simulink library "outp"  (R2021b)
settings: Solver=VariableStepAuto  StartTime=0.0  StopTime=10.0  RelTol=1e-3
undefined symbols (not defined in the file or in its folder): ENUM_PMMMODE_CHARGE, ENUM_PMMMODE_IDLE, ENUM_PMMMODE_INITIALIZE, ENUM_PMMMODE_POWERDOWN, ENUM_PMMMODE_SLEEP, FALSE, Left, outp, slcm, TRUE
libraries: FVT_lib x956, hcu_lib x4, simulink x1
(part 5 of 10)

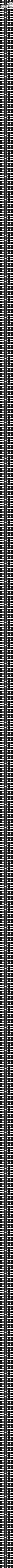
== system outp/OUTP/outpmodule ==
  VACC_EACEnDemand_enum : Inport
  VACC_CACTempOverHigh_flg : Inport  Port=2
  VACC_CACPresWarn_flg : Inport  Port=3
  VACC_CACPresReady_flg : Inport  Port=4
  VACC_EHPSEnDemand_enum : Inport  Port=5
  VACC_CACOverrun_flg : Inport  Port=6
  VACC_CACRunFail_flg : Inport  Port=7
  VACC_EHPSMotorDemSpd_rpm : Inport  Port=8
  VACC_EHPSSpdDemTimeout_flg : Inport  Port=9
  VACC_EHPSEnTimeout_flg : Inport  Port=10
  VACC_EHPSDisEnTimeout_flg : Inport  Port=11
  VACC_DCDCEnDemamd_enum : Inport  Port=12
  VACC_EHPSSpdCtrlMode_enum : Inport  Port=13
  VACC_EACSpdDemand_rpm : Inport  Port=14
  VACC_CACFanReq_flg : Inport  Port=15
  VAPM_VehSpeed_kph : Inport  Port=16
  VAPM_VehSpeedTimeOut_flg : Inport  Port=17
  VAPM_FSOffSw_enum : Inport  Port=18
  VAPM_FSOffSwTimeOut_flg : Inport  Port=19
  VAPM_ChrgPlugSta_enum : Inport  Port=20
  VAPM_PASDRMR_cm : Inport  Port=21
  VAPM_PASDRML_cm : Inport  Port=22
  VAPM_PASDRCR_cm : Inport  Port=23
  VAPM_PASDRCL_cm : Inport  Port=24
  VAPM_PASDFMR_cm : Inport  Port=25
  VAPM_PASDFML_cm : Inport  Port=26
  VAPM_PASDFCR_cm : Inport  Port=27
  VAPM_PASDFCL_cm : Inport  Port=28
  VAPM_APSDRLR_cm : Inport  Port=29
  VAPM_APSDRLL_cm : Inport  Port=30
  VAPM_APSDFLR_cm : Inport  Port=31
  VAPM_APSDFLL_cm : Inport  Port=32
  VAPM_PASAFCL_enum : Inport  Port=33
  VAPM_PASARMR_enum : Inport  Port=34
  VAPM_PASARML_enum : Inport  Port=35
  VAPM_PASARCR_enum : Inport  Port=36
  VAPM_PASARCL_enum : Inport  Port=37
  VAPM_PASAFMR_enum : Inport  Port=38
  VAPM_PASAFML_enum : Inport  Port=39
  VAPM_PASAFCR_enum : Inport  Port=40
  VAPM_USSStaRMR_flg : Inport  Port=41
  VAPM_USSStaRML_flg : Inport  Port=42
  VAPM_USSStaRLR_flg : Inport  Port=43
  VAPM_USSStaRLL_flg : Inport  Port=44
  VAPM_USSStaRCR_flg : Inport  Port=45
  VAPM_USSStaRCL_flg : Inport  Port=46
  VAPM_USSStaFMR_flg : Inport  Port=47
  VAPM_USSStaFML_flg : Inport  Port=48
  VAPM_USSStaFLR_flg : Inport  Port=49
  VAPM_USSStaFLL_flg : Inport  Port=50
  VAPM_USSStaFCR_flg : Inport  Port=51
  VAPM_USSStaFCL_flg : Inport  Port=52
  VAPM_Chime_enum : Inport  Port=53
  VAPM_SNSRLayout_enum : Inport  Port=54
  VAPM_StaFSya_flg : Inport  Port=55
  VAPM_ModOperation_enum : Inport  Port=56
  VAPM_BrkPedalPos_pct : Inport  Port=57
  VAPM_BrkPedalPosTimeOut_flg : Inport  Port=58
  VAPM_LFRawWhlSpeed_kph : Inport  Port=59
  VAPM_LFRawWhlSpeedTimeOut_flg : Inport  Port=60
  VAPM_RFRawWhlSpeed_kph : Inport  Port=61
  VAPM_RFRawWhlSpeedTimeOut_flg : Inport  Port=62
  VAPM_LRRawWhlSpeed_kph : Inport  Port=63
  VAPM_LRRawWhlSpeedTimeOut_flg : Inport  Port=64
  VAPM_RRRawWhlSpeed_kph : Inport  Port=65
  VAPM_RRRawWhlSpeedTimeOut_flg : Inport  Port=66
  VAPM_LFRawWhlSpeedV_flg : Inport  Port=67
  VAPM_LFRawWhlSpeedVTimeOut_flg : Inport  Port=68
  VAPM_RFRawWhlSpeedV_flg : Inport  Port=69
  VAPM_RFRawWhlSpeedVTimeOut_flg : Inport  Port=70
  VAPM_LRRawWhlSpeedV_flg : Inport  Port=71
  VAPM_LRRawWhlSpeedVTimeOut_flg : Inport  Port=72
  VAPM_RRRawWhlSpeedV_flg : Inport  Port=73
  VAPM_RRRawWhlSpeedVTimeOut_flg : Inport  Port=74
  VAPM_LFWhlRotDir_enum : Inport  Port=75
  VAPM_LFWhlRotDirTimeOut_flg : Inport  Port=76
  VAPM_RFWhlRotDir_enum : Inport  Port=77
  VAPM_RFWhlRotDirTimeOut_flg : Inport  Port=78
  VAPM_LRWhlRotDir_enum : Inport  Port=79
  VAPM_LRWhlRotDirTimeOut_flg : Inport  Port=80
  VAPM_RRWhlRotDir_enum : Inport  Port=81
  VAPM_RRWhlRotDirTimeOut_flg : Inport  Port=82
  VAPM_LFPulseCountV_flg : Inport  Port=83
  VAPM_LFPulseCountVTimeOut_flg : Inport  Port=84
  VAPM_RFPulseCountV_flg : Inport  Port=85
  VAPM_RFPulseCountVTimeOut_flg : Inport  Port=86
  VAPM_LRPulseCountV_flg : Inport  Port=87
  VAPM_LRPulseCountVTimeOut_flg : Inport  Port=88
  VAPM_RRPulseCountV_flg : Inport  Port=89
  VAPM_RRPulseCountVTimeOut_flg : Inport  Port=90
  VAPM_LFPulseCount_enum : Inport  Port=91
  VAPM_LFPulseCountTimeOut_flg : Inport  Port=92
  VAPM_RFPulseCount_enum : Inport  Port=93
  VAPM_RFPulseCountTimeOut_flg : Inport  Port=94
  VAPM_LRPulseCount_enum : Inport  Port=95
  VAPM_LRPulseCountTimeOut_flg : Inport  Port=96
  VAPM_RRPulseCount_enum : Inport  Port=97
  VAPM_RRPulseCountTimeOut_flg : Inport  Port=98
  VAPM_ShifterHandleCmd_enum : Inport  Port=99
  VAPM_ShifterHandleCmdTimeOut_flg : Inport  Port=100
  VAPM_DriIntend_enum : Inport  Port=101
  VAPM_DriIntendTimeOut_flg : Inport  Port=102
  VAPM_EPSAOIControl_enum : Inport  Port=103
  VAPM_EPSAOIControlTimeOut_flg : Inport  Port=104
  VAPM_SASAngle_Deg : Inport  Port=105
  VAPM_SASAngleTimeOut_flg : Inport  Port=106
  VAPM_SASSpeed_degps : Inport  Port=107
  VAPM_SASSpeedTimeOut_flg : Inport  Port=108
  VAPM_SASSpeedValid_flg : Inport  Port=109
  VAPM_SASSpeedValidTimeOut_flg : Inport  Port=110
  VAPM_SASCAL_flg : Inport  Port=111
  VAPM_SASCALTimeOut_flg : Inport  Port=112
  VAPM_SASV_flg : Inport  Port=113
  VAPM_SASVTimeOut_flg : Inport  Port=114
  VAPM_GRADE_Deg : Inport  Port=115
  VAPM_GRADETimeOut_flg : Inport  Port=116
  VAPM_YawRate_degps : Inport  Port=117
  VAPM_YawRateTimeOut_flg : Inport  Port=118
  VAPM_LatAccel_Gps : Inport  Port=119
  VAPM_LatAccelTimeOut_flg : Inport  Port=120
  VAPM_LongAccel_Gps : Inport  Port=121
  VAPM_LongAccelTimeOut_flg : Inport  Port=122
  VAPM_MCPressure_bar : Inport  Port=123
  VAPM_MCPressureTimeOut_flg : Inport  Port=124
  VAPM_YawRateV_flg : Inport  Port=125
  VAPM_YawRateVTimeOut_flg : Inport  Port=126
  VAPM_LatAccelV_flg : Inport  Port=127
  VAPM_LatAccelVTimeOut_flg : Inport  Port=128
  VAPM_LongAccelV_flg : Inport  Port=129
  VAPM_LongAccelVTimeOut_flg : Inport  Port=130
  VAPM_MCPressureV_bar : Inport  Port=131
  VAPM_MCPressureVTimeOut_flg : Inport  Port=132
  VAPM_BrkSwSta_flg : Inport  Port=133
  VAPM_BrkSwStaTimeOut_flg : Inport  Port=134
  VAPM_BrkSwV_flg : Inport  Port=135
  VAPM_BrkSwVTimeOut_flg : Inport  Port=136
  VAPM_ESCStandstill_flg : Inport  Port=137
  VAPM_ESCStandstillTimeOut_flg : Inport  Port=138
  VAPM_ESCAPSSta_enum : Inport  Port=139
  VAPM_ESCAPSStaTimeOut_flg : Inport  Port=140
  VAPM_EPBExtReleaseAvail_flg : Inport  Port=141
  VAPM_EPBExtReleaseAvailTimeOut_flg : Inport  Port=142
  VAPM_EPBExtApplyAvail_flg : Inport  Port=143
  VAPM_EPBExtApplyAvailTimeOut_flg : Inport  Port=144
  VAPM_EPBErrSta_enum : Inport  Port=145
  VAPM_EPBErrStaTimeOut_flg : Inport  Port=146
  VAPM_EPBSta_enum : Inport  Port=147
  VAPM_EPBStaTimeOut_flg : Inport  Port=148
  VAPM_AVMparkingcancel_enum : Inport  Port=149
  VAPM_AVMparkingcancelTimeOut_flg : Inport  Port=150
  VAPM_AVMparkingexcute_enum : Inport  Port=151
  VAPM_AVMparkingexcuteTimeOut_flg : Inport  Port=152
  VAPM_AVMParkingmode_enum : Inport  Port=153
  VAPM_AVMParkingmodeTimeOut_flg : Inport  Port=154
  VAPM_AVMErrSTA_flg : Inport  Port=155
  VAPM_AVMErrSTATimeOut_flg : Inport  Port=156
  VAPM_IVIStatus_flg : Inport  Port=157
  VAPM_IVIStatusTimeOut_flg : Inport  Port=158
  VAPM_CAASSw_enum : Inport  Port=159
  VAPM_CAASSwTimeOut_flg : Inport  Port=160
  VAPM_IVIScreen_enum : Inport  Port=161
  VAPM_IVIScreenTimeOut_flg : Inport  Port=162
  VAPM_ABSActive_flg : Inport  Port=163
  VAPM_ABSActiveTimeOut_flg : Inport  Port=164
  VAPM_TCSActive_flg : Inport  Port=165
  VAPM_TCSActiveTimeOut_flg : Inport  Port=166
  VAPM_DriverSeatBeltCmd_flg : Inport  Port=167
  VAPM_DriverSeatBeltCmdTimeOut_flg : Inport  Port=168
  VAPM_APSProgressPCT_pct : Inport  Port=169
  VAPM_APSRQDisplay_enum : Inport  Port=170
  VAPM_APSSWVer_enum : Inport  Port=171
  VAPM_APSHWVer_enum : Inport  Port=172
  VAPM_APSExitCondition_enum : Inport  Port=173
  VAPM_APSAngleTarget_Deg : Inport  Port=174
  VAPM_APSVRqEPASCtrl_flg : Inport  Port=175
  VAPM_APSRqEPASCtrl_flg : Inport  Port=176
  VAPM_CAASSta_enum : Inport  Port=177
  VAPM_DKCPDkeyAreaRAPSSta_enum : Inport  Port=178
  VAPM_DKCParkingModeCmd_enum : Inport  Port=179
  VAPM_PUIDLowPower_flg : Inport  Port=180
  VAPM_CAASVMCReqA_flg : Inport  Port=181
  VAPM_APSShiftPosnReq_enum : Inport  Port=182
  VAPM_APSSpeedCMD_kph : Inport  Port=183
  VAPM_APSVMCReqA_flg : Inport  Port=184
  VAPM_RAPSBCMLamp_enum : Inport  Port=185
  VAPM_RAPSBCMLockReq_flg : Inport  Port=186
  VAPM_APSPwrReq_enum : Inport  Port=187
  VAPM_RAPSErrWarnSta_enum : Inport  Port=188
  VAPM_RAPSErrLv1_flg : Inport  Port=189
  VAPM_IVIUserTakeOverAPSSta_flg : Inport  Port=190
  VBCM_FDCBCMLBeamCmd_flg : Inport  Port=191
  VBCM_FDCBCMPLampCmd_flg : Inport  Port=192
  VBCM_FDCBCMHBeamCmd_flg : Inport  Port=193
  VBCM_FDCBCMSMKLCmd_flg : Inport  Port=194
  VBCM_FDCBCMSMKRCmd_flg : Inport  Port=195
  VBCM_FDCBCMDVRSignalLCmd_flg : Inport  Port=196
  VBCM_FDCBCMDVRSignalRCmd_flg : Inport  Port=197
  VBCM_FDCBCMBSDBuzzerCmd_flg : Inport  Port=198
  VBCM_FDCBCMSLTLpCmd_flg : Inport  Port=199
  VBCM_FDCBCMSRTLpCmd_flg : Inport  Port=200
  VBCM_FDCBCMLTurnLpCmd_flg : Inport  Port=201
  VBCM_FDCBCMRTurnLpCmd_flg : Inport  Port=202
  VBCM_FDCBCMStopINDCmd_flg : Inport  Port=203
  VBCM_FDCBCMSTOPBALLCmd_flg : Inport  Port=204
  VBCM_FDCBCMInnerCallBellCmd_flg : Inport  Port=205
  VBCM_FDCBCMCallBellCmd_flg : Inport  Port=206
  VBCM_FDCBCMWiperHCmd_flg : Inport  Port=207
  VBCM_FDCBCMWasherCmd_flg : Inport  Port=208
  VBCM_FDCBCMWiperLCmd_flg : Inport  Port=209
  VBCM_FDCBCMLDRLCmd_flg : Inport  Port=210
  VBCM_FDCBCMRDRLCmd_flg : Inport  Port=211
  VBCM_FDCBCMRFLampCmd_flg : Inport  Port=212
  VBCM_TurnLpPatternSta_enum : Inport  Port=213
  VBCM_FDCBCMFDoorSta_flg : Inport  Port=214
  VBCM_FDCBCMMDoorSta_flg : Inport  Port=215
  VBCM_FDCBCMRDoorSta_flg : Inport  Port=216
  VBCM_FDCBCMRoomLpAmbCmd_flg : Inport  Port=217
  VBCM_FDCBCMLBSDRCmd_flg : Inport  Port=218
  VBCM_FDCBCMLBSDYCmd_flg : Inport  Port=219
  VBCM_FDCBCMRBSDRCmd_flg : Inport  Port=220
  VBCM_FDCBCMRBSDYCmd_flg : Inport  Port=221
  VBCM_FDCBCMEmExitSWSta_flg : Inport  Port=222
  VBCM_InnerBuzzerModeSta_enum : Inport  Port=223
  VBCM_FDCBCMInnerBuzzerCmd_flg : Inport  Port=224
  VBCM_FDCBCMRoomLpAmbSetSta_flg : Inport  Port=225
  VBCM_FDCBCMRoomLpSetSta_flg : Inport  Port=226
  VBCM_FDCBCMFRoomLpSetSta_pct : Inport  Port=227
  VBCM_FDCBCMFRoomLpCmd_pct : Inport  Port=228
  VBCM_FDCBCMMRoomLpSetSta_pct : Inport  Port=229
  VBCM_FDCBCMMRoomLpCmd_pct : Inport  Port=230
  VBCM_FDCBCMRRoomLpSetSta_pct : Inport  Port=231
  VBCM_FDCBCMRRoomLpCmd_pct : Inport  Port=232
  VBCM_FDCBCMHelpINDCmd_flg : Inport  Port=233
  VBCM_FDCBCMOSDrOpenSWSta_enum : Inport  Port=234
  VBCM_FDCBCMEmSVCmd_flg : Inport  Port=235
  VBCM_FDCBCMFDOpenSVCmd_flg : Inport  Port=236
  VBCM_FDCBCMFDCloseSVCmd_flg : Inport  Port=237
  VBCM_FDCBCMMDOpenSVCmd_flg : Inport  Port=238
  VBCM_FDCBCMMDCloseSVCmd_flg : Inport  Port=239
  VBCM_FDCBCMLTurnSWSta_flg : Inport  Port=240
  VBCM_FDCBCMRTurnSWSta_flg : Inport  Port=241
  VBCM_FDCBCMRGearSta_flg : Inport  Port=242
  VBCM_FDCBCMBrakeCmd_flg : Inport  Port=243
  VBCM_FDCBCMTurnBuzzerENSta_flg : Inport  Port=244
  VBCM_WakeUp_flg : Inport  Port=245
  VBCM_KeepWakeUp_flg : Inport  Port=246
  VDDM_C3BMS6RCDTC_raw32 : Inport  Port=247
  VDDM_C3BMS6CSDTC_raw32 : Inport  Port=248
  VDDM_C3BMS6LCDTC_raw32 : Inport  Port=249
  VDDM_C3BMS1RCDTC_raw32 : Inport  Port=250
  VDDM_C3BMS1CSDTC_raw32 : Inport  Port=251
  VDDM_C3BMS1LCDTC_raw32 : Inport  Port=252
  VDDM_C3CCU1RCDTC_raw32 : Inport  Port=253
  VDDM_C3CCU1CSDTC_raw32 : Inport  Port=254
  VDDM_C3CCU1LCDTC_raw32 : Inport  Port=255
  VDDM_C3CCU2RCDTC_raw32 : Inport  Port=256
  VDDM_C3CCU2CSDTC_raw32 : Inport  Port=257
  VDDM_C3CCU2LCDTC_raw32 : Inport  Port=258
  VDDM_C1ABM1RCDTC_raw32 : Inport  Port=259
  VDDM_C1ABM1CSDTC_raw32 : Inport  Port=260
  VDDM_C1ABM1LCDTC_raw32 : Inport  Port=261
  VDDM_Lv1ErrDTC_raw32 : Inport  Port=262
  VDDM_Lv2ErrDTC_raw32 : Inport  Port=263
  VDDM_Lv3ErrDTC_raw32 : Inport  Port=264
  VDDM_Lv4ErrDTC_raw32 : Inport  Port=265
  VDDM_BrkSWErrDTC_raw32 : Inport  Port=266
  VDDM_BrkSWNoBacDTC_raw32 : Inport  Port=267
  VDDM_KeyAuthDTC_raw32 : Inport  Port=268
  VDDM_ONtoRdyDTC_raw32 : Inport  Port=269
  VDDM_HVB4PreDTC_raw32 : Inport  Port=270
  VDDM_MCU4PreDTC_raw32 : Inport  Port=271
  VDDM_DCDC4PreDTC_raw32 : Inport  Port=272
  VDDM_HVRlyCloDTC_raw32 : Inport  Port=273
  VDDM_BMSRdyDTC_raw32 : Inport  Port=274
  VDDM_DCDCEnaDTC_raw32 : Inport  Port=275
  VDDM_HiLvSaChkDTC_raw32 : Inport  Port=276
  VDDM_MidLvSaChkDTC_raw32 : Inport  Port=277
  VDDM_MCUDisDTC_raw32 : Inport  Port=278
  VDDM_DCDCDisDTC_raw32 : Inport  Port=279
  VDDM_HVRlyOpDTC_raw32 : Inport  Port=280
  VDDM_MCUActDTC_raw32 : Inport  Port=281
  VDDM_OBC4PreDTC_raw32 : Inport  Port=282
  VDDM_IniLVLoDTC_raw32 : Inport  Port=283
  VDDM_LVSupLoDTC_raw32 : Inport  Port=284
  VDDM_LVSupHiDTC_raw32 : Inport  Port=285
  VDDM_DrStSWDTC_raw32 : Inport  Port=286
  VDDM_FLDoorSWDTC_raw32 : Inport  Port=287
  VDDM_RLDoorSWDTC_raw32 : Inport  Port=288
  VDDM_FRDoorSWDTC_raw32 : Inport  Port=289
  VDDM_RRDoorSWDTC_raw32 : Inport  Port=290
  VDDM_HoodSWDTC_raw32 : Inport  Port=291
  VDDM_TailgaSWDTC_raw32 : Inport  Port=292
  VDDM_EDriveSysErrVCUErr_flg : Inport  Port=293
  VDDM_VehMalfunLevel_enum : Inport  Port=294
  VDDM_APS1SigOoRDTC_raw32 : Inport  Port=295
  VDDM_APS2SigOoRDTC_raw32 : Inport  Port=296
  VDDM_APSCorrErrDTC_raw32 : Inport  Port=297
  VDDM_MCUF1NoComDTC_raw32 : Inport  Port=298
  VDDM_MCUR1NoComDTC_raw32 : Inport  Port=299
  VDDM_Shifter1NoComDTC_raw32 : Inport  Port=300
  VDDM_ESC7NoComDTC_raw32 : Inport  Port=301
  VDDM_ESC1NoComDTC_raw32 : Inport  Port=302
  VDDM_ESC5NoComDTC_raw32 : Inport  Port=303
  VDDM_EnterNewOperCyc_flg : Inport  Port=304
  VDDM_DiagHCrashDTC_raw32 : Inport  Port=305
  VDDM_DiagFLTSDTC_raw32 : Inport  Port=306
  VDDM_DiagFRTSDTC_raw32 : Inport  Port=307
  VDDM_DiagRLTSDTC_raw32 : Inport  Port=308
  VDDM_DiagRRTSDTC_raw32 : Inport  Port=309
  VDDM_FCLUSSDTC_raw32 : Inport  Port=310
  VDDM_FMLUSSDTC_raw32 : Inport  Port=311
  VDDM_FMRUSSDTC_raw32 : Inport  Port=312
  VDDM_FCRUSSDTC_raw32 : Inport  Port=313
  VDDM_RCLUSSDTC_raw32 : Inport  Port=314
  VDDM_RMLUSSDTC_raw32 : Inport  Port=315
  VDDM_RMRUSSDTC_raw32 : Inport  Port=316
  VDDM_RCRUSSDTC_raw32 : Inport  Port=317
  VDDM_FLLUSSDTC_raw32 : Inport  Port=318
  VDDM_FLRUSSDTC_raw32 : Inport  Port=319
  VDDM_RLLUSSDTC_raw32 : Inport  Port=320
  VDDM_RLRUSSDTC_raw32 : Inport  Port=321
  VDDM_FCM2NoComDTC_raw32 : Inport  Port=322
  VDDM_FCM2RCErrDTC_raw32 : Inport  Port=323
  VDDM_FCM2CSErrDTC_raw32 : Inport  Port=324
  VDDM_FCM3NoComDTC_raw32 : Inport  Port=325
  VDDM_FCM3RCErrDTC_raw32 : Inport  Port=326
  VDDM_FCM3CSErrDTC_raw32 : Inport  Port=327
  VDDM_FCM4NoComDTC_raw32 : Inport  Port=328
  VDDM_FCM4CSErrDTC_raw32 : Inport  Port=329
  VDDM_FCM5NoComDTC_raw32 : Inport  Port=330
  VDDM_FCM5CSErrDTC_raw32 : Inport  Port=331
  VDDM_ZoneSCPNoComDTC_raw32 : Inport  Port=332
  VDDM_BMSSigErrDetDTC_raw32 : Inport  Port=333
  VDDM_FCMACCSigErrDetDTC_raw32 : Inport  Port=334
  VDDM_FrMCUSigErrDetDTC_raw32 : Inport  Port=335
  VDDM_RrMCUSigErrDetDTC_raw32 : Inport  Port=336
  VDDM_CCUSigErrDetDTC_raw32 : Inport  Port=337
  VDDM_ACCAccelCmdErrDetDTC_raw32 : Inport  Port=338
  VDDM_ACCMalfuncDetDTC_raw32 : Inport  Port=339
  VDDM_CCMalfuncDetDTC_raw32 : Inport  Port=340
  VDDM_MSAMalfuncDetDTC_raw32 : Inport  Port=341
  VDDM_ISAMalfuncDetDTC_raw32 : Inport  Port=342
  VDDM_MCUF1RCErrDTC_raw32 : Inport  Port=343
  VDDM_MCUR1RCErrDTC_raw32 : Inport  Port=344
  VDDM_MCUF1CSErrDTC_raw32 : Inport  Port=345
  VDDM_MCUR1CSErrDTC_raw32 : Inport  Port=346
  VDDM_Shifter1RCErrDTC_raw32 : Inport  Port=347
  VDDM_Shifter1CSErrDTC_raw32 : Inport  Port=348
  VDDM_ESC7RCErrDTC_raw32 : Inport  Port=349
  VDDM_ESC7CSErrDTC_raw32 : Inport  Port=350
  VDDM_ESC1RCErrDTC_raw32 : Inport  Port=351
  VDDM_ESC1CSErrDTC_raw32 : Inport  Port=352
  VDDM_ESC5RCErrDTC_raw32 : Inport  Port=353
  VDDM_ESC5CSErrDTC_raw32 : Inport  Port=354
  VDDM_FrMCUTqErrDTC_raw32 : Inport  Port=355
  VDDM_RrMCUTqErrDTC_raw32 : Inport  Port=356
  VDDM_LFBatwarnDTC_raw32 : Inport  Port=357
  VDDM_RFBatwarnDTC_raw32 : Inport  Port=358
  VDDM_LRBatwarnDTC_raw32 : Inport  Port=359
  VDDM_RRBatwarnDTC_raw32 : Inport  Port=360
  VDDM_LFPressIndiDTC_raw32 : Inport  Port=361
  VDDM_RFPressIndiDTC_raw32 : Inport  Port=362
  VDDM_LRPressIndiDTC_raw32 : Inport  Port=363
  VDDM_RRPressIndiDTC_raw32 : Inport  Port=364
  VDDM_LFWheelTmpHighDTC_raw32 : Inport  Port=365
  VDDM_RFWheelTmpHighDTC_raw32 : Inport  Port=366
  VDDM_LRWheelTmpHighDTC_raw32 : Inport  Port=367
  VDDM_RRWheelTmpHighDTC_raw32 : Inport  Port=368
  VDDM_LFSensorFailDTC_raw32 : Inport  Port=369
  VDDM_RFSensorFailDTC_raw32 : Inport  Port=370
  VDDM_LRSensorFailDTC_raw32 : Inport  Port=371
  VDDM_RRSensorFailDTC_raw32 : Inport  Port=372
  VDDM_C1EPAS2LCDTC_raw32 : Inport  Port=373
  VDDM_5vAPS1PwrErrDTC_raw32 : Inport  Port=374
  VDDM_5vAPS2PwrErrDTC_raw32 : Inport  Port=375
  VDDM_EPBLockTODTC_raw32 : Inport  Port=376
  VDDM_EPBUnlockTODTC_raw32 : Inport  Port=377
  VDDM_LimpHomeActTmp_flg : Inport  Port=378
  VDDM_DTCDetect_enum : Inport  Port=379
  VDDM_EngagePFail_flg : Inport  Port=380
  VDDM_DisengagePFail_flg : Inport  Port=381
  VDDM_VCURAPSErrLv2_flg : Inport  Port=382
  VDDM_VCURAPSErrLv3_flg : Inport  Port=383
  VDDM_EDriveSysErrShifterErr_flg : Inport  Port=384
  VDDM_LVSysErrPwrOutErr_flg : Inport  Port=385
  VDDM_HVRlyOpFail_flg : Inport  Port=386
  VDDM_MCUActDisFail_flg : Inport  Port=387
  VDDM_VCUBrkSWSta_enum : Inport  Port=388
  VDDM_VCUFLDoorSta_flg : Inport  Port=389
  VDDM_VCUFRDoorSta_flg : Inport  Port=390
  VDDM_VCURLDoorSta_flg : Inport  Port=391
  VDDM_VCURRDoorSta_flg : Inport  Port=392
  VDDM_SysAllowReadySta_flg : Inport  Port=393
  VDDM_VCUHoodSWSta_flg : Inport  Port=394
  VDDM_VCUTailgateSWSta_flg : Inport  Port=395
  VDHP_ActAPSPosn_pct : Inport  Port=396
  VDHP_EAPS1MIN_pct : Inport  Port=397
  VDHP_EAPS2MIN_pct : Inport  Port=398
  VDHP_ResetPedalZeroPosStart_flg : Inport  Port=399
  VDHP_EAPS1NRM_pct : Inport  Port=400
  VDHP_EAPS2NRM_pct : Inport  Port=401
  VDID_VSS_kph : Inport  Port=402
  VDID_RUNTM_s : Inport  Port=403
  VDID_MILDIST_km : Inport  Port=404
  VDID_WARMUPS_cnt : Inport  Port=405
  VDID_CLRDIST_km : Inport  Port=406
  VDID_APPD_pct : Inport  Port=407
  VDID_APPE_pct : Inport  Port=408
  VDID_MILTIME_min : Inport  Port=409
  VDID_CLRTIME_min : Inport  Port=410
  VDID_BATSOC_pct : Inport  Port=411
  VDID_HEVBATT_V : Inport  Port=412
  VDID_ODOMETER_km : Inport  Port=413
  VDID_BATSOH_pct : Inport  Port=414
  VDID_HVBCellVoltMin_V : Inport  Port=415
  VDID_HVBCellVoltMax_V : Inport  Port=416
  VDID_HVESSCHARGELIM_kW : Inport  Port=417
  VDID_HVESSCHARGEACT_kW : Inport  Port=418
  VDID_HVESSENER_Whps : Inport  Port=419
  VDID_NUMPSATRIPSFLTMEMCLR_cnt : Inport  Port=420
  VDID_HVBattCurr_Ahps : Inport  Port=421
  VDID_PSAR_sec : Inport  Port=422
  VDID_PSAL_sec : Inport  Port=423
  VDID_IPSAR_sec : Inport  Port=424
  VDID_IPSAL_sec : Inport  Port=425
  VDID_CPSAR_sec : Inport  Port=426
  VDID_CPSAL_sec : Inport  Port=427
  VDID_HVBNAH_Ahr : Inport  Port=428
  VDID_HVBNE_kWh : Inport  Port=429
  VDID_IGNCNTR_cnt : Inport  Port=430
  VDID_TNBCPSAR_Ahr : Inport  Port=431
  VDID_TNBCPSAL_Ahr : Inport  Port=432
  VDID_TNECPSAR_kWh : Inport  Port=433
  VDID_TNECPSAL_kWh : Inport  Port=434
  VDID_TEBPSAR_kWh : Inport  Port=435
  VDID_TEBPSAL_kWh : Inport  Port=436
  VDID_TGEOVCR_kWh : Inport  Port=437
  VDID_TGEOVCL_kWh : Inport  Port=438
  VDID_GECHGOVCDCR_kWh : Inport  Port=439
  VDID_GECHGOVCDCL_kWh : Inport  Port=440
  VDID_GECHGOVCACR_kWh : Inport  Port=441
  VDID_GECHGOVCACL_kWh : Inport  Port=442
  VDID_RESSV2XENNONPSAR_kWh : Inport  Port=443
  VDID_RESSV2XENNONPSAL_kWh : Inport  Port=444
  VDID_PKER_kphsqr : Inport  Port=445
  VDID_PKEL_kphsqr : Inport  Port=446
  VDID_ResetCDEODTR_km : Inport  Port=447
  VDID_CDEODTR_km : Inport  Port=448
  VDID_CDEODTL_km : Inport  Port=449
  VDID_AvgBattTempPSAR_C : Inport  Port=450
  VDID_AvgBattTempPSAL_C : Inport  Port=451
  VDID_AvgBattTempOVCR_C : Inport  Port=452
  VDID_AvgBattTempOVCL_C : Inport  Port=453
  VDID_AvgBattTempOFFR_C : Inport  Port=454
  VDID_AvgBattTempOFFL_C : Inport  Port=455
  VDID_QTYPSATRIPSR_cnt : Inport  Port=456
  VDID_QTYPSATRIPSL_cnt : Inport  Port=457
  VDID_RESSCNTDODRNGR_cnt : Inport  Port=458
  VDID_RESSCNTDODRNGL_cnt : Inport  Port=459
  VDID_ETMATOER_kWh : Inport  Port=460
  VDID_ETMATOEL_kWh : Inport  Port=461
  VDID_ETMBTOER_kWh : Inport  Port=462
  VDID_ETMBTOEL_kWh : Inport  Port=463
  VDID_RESSTIMESOCPSARNGR_s : Inport  Port=464
  VDID_RESSTIMESOCPSARNGL_s : Inport  Port=465
  VDID_RESSTIMESOCCHGRNGR_s : Inport  Port=466
  VDID_RESSTIMESOCCHGRNGL_s : Inport  Port=467
  VDID_RESSTIMESOCOFFRNGR_s : Inport  Port=468
  VDID_RESSTIMESOCOFFRNGL_s : Inport  Port=469
  VDID_MAXBATTEMPL_C : Inport  Port=470
  VDID_MINBATTEMPL_C : Inport  Port=471
  VDID_AVGBATTEMPL_C : Inport  Port=472
  VDID_PROTOCOLID_enum : Inport  Port=473
  VDID_RESSTTEMPRNGAXIS_enum : Inport  Port=474
  VDID_RESSTIMESOCRNGAXIS_enum : Inport  Port=475
  VDID_RESSCNTSDODRNGAXIS_enum : Inport  Port=476
  VDID_CALID_cnt : Inport  Port=477
  VDID_ECUNAME_cnt : Inport  Port=478
  VDID_PKERNumerator_kphsqr : Inport  Port=479
  VDID_PKELNumerator_kphsqr : Inport  Port=480
  VDID_BattTempPSAR_sec : Inport  Port=481
  VDID_BattTempPSAL_sec : Inport  Port=482
  VDID_OVCR_sec : Inport  Port=483
  VDID_OVCL_sec : Inport  Port=484
  VDID_OFFR_sec : Inport  Port=485
  VDID_OFFL_sec : Inport  Port=486
  VDID_AVGBATTEMPL_sec : Inport  Port=487
  VDID_VinCode_cnt : Inport  Port=488
  VDID_STASUP_enum : Inport  Port=489
  VDID_HEVMODE_enum : Inport  Port=490
  VDID_HVBATT_A : Inport  Port=491
  VDID_DIDModelVersion_raw : Inport  Port=492
  VDID_DIDModelVersionChksum_raw : Inport  Port=493
  VDKC_DKCTimeSN_cnt : Inport  Port=494
  VDKC_DKCAuthSta_enum : Inport  Port=495
  VDKC_TimeSNDKCFbk_cnt : Inport  Port=496
  VDKC_KeyMissSta_flg : Inport  Port=497
  VDKC_KeyModeSta_enum : Inport  Port=498
  VDKC_DkeyShowIVISta_enum : Inport  Port=499
  VDKC_KeyAreaPS_enum : Inport  Port=500
  VDKC_KeyAreaLockUnlock_enum : Inport  Port=501
  VDKC_PCommandToBCM_enum : Inport  Port=502
  VDKC_DKeyWelcomeSta_enum : Inport  Port=503
  VDKC_KeyAreaPTG_enum : Inport  Port=504
  VDKC_KeyAreaSPTGSta_enum : Inport  Port=505
  VDKC_UIDLowPowerSta_enum : Inport  Port=506
  VDKC_DkeyAreaRAPSSta_enum : Inport  Port=507
  VDKC_ParkingModeCmd_enum : Inport  Port=508
  VDKC_KeyNumSta_enum : Inport  Port=509
  VDKC_KeyTypeSta_enum : Inport  Port=510
  VDKC_FDCDKCAllowSleep_flg : Inport  Port=511
  VDKC_JudgeKeepUnlockZone_flg : Inport  Port=512
  VDSC_DISCTurn_flg : Inport  Port=513
  VDSC_DISCTargetSpd_kph : Inport  Port=514
  VDSC_DISCSta_enum : Inport  Port=515
  VDSC_DISCButtSta_flg : Inport  Port=516
  VNMM_AllCANTxReq_flg : Inport  Port=517
  VNMM_NMmTxReq_flg : Inport  Port=518
  VNMM_Awake_enum : Inport  Port=519
  VNMM_CSB_flg : Inport  Port=520
  VNMM_ErrorState_enum : Inport  Port=521
  VNMM_NodeID_enum : Inport  Port=522
  VNMM_PNI_flg : Inport  Port=523
  VNMM_RptMsgReq_flg : Inport  Port=524
  VNMM_WakeUp_enum : Inport  Port=525
  VNMM_ActiveWU_flg : Inport  Port=526
  VNMM_SysNMmSta_enum : Inport  Port=527
  VNMM_NetworkReq_flg : Inport  Port=528
  VPMM_SysPowerMode_enum : Inport  Port=529
  VPMM_PowerUpState_enum : Inport  Port=530
  VPMM_PowerDownState_enum : Inport  Port=531
  VPMM_ChrgState_enum : Inport  Port=532
  VPMM_PowerUpFault_enum : Inport  Port=533
  VPMM_PowerDownFault_enum : Inport  Port=534
  VPMM_ChrgFault_enum : Inport  Port=535
  VPMM_IRCRlyClose_flg : Inport  Port=536
  VPMM_IGNRlyClose_flg : Inport  Port=537
  VPMM_BattHVDem_enum : Inport  Port=538
  VPMM_DCDCRlyDem_enum : Inport  Port=539
  VPMM_CACRlyDem_enum : Inport  Port=540
  VPMM_MCUHVLoopDem_enum : Inport  Port=541
  VPMM_EHPSRlyDem_enum : Inport  Port=542
  VPMM_ACHVLoopDem_enum : Inport  Port=543
  VPMM_HVSysReady_enum : Inport  Port=544
  VPMM_DrivelineRelease_enum : Inport  Port=545
  VPMM_ActiveDischargeReq_enum : Inport  Port=546
  VPMM_VCUMCUEn_flg : Inport  Port=547
  VPMM_VCUMCUFailRst_flg : Inport  Port=548
  VPMM_HVILFail_flg : Inport  Port=549
  VPMM_LostHVComActivePwrDown_flg : Inport  Port=550
  VPMM_LVBattLowInd_enum : Inport  Port=551
  VPMM_ChrgPowerUpFail_flg : Inport  Port=552
  VPMM_ChrgBCUHVFail_flg : Inport  Port=553
  VPMM_HVFailureChkPass_flg : Inport  Port=554
  VPMM_HVILDetectFail_flg : Inport  Port=555
  VPMM_V2BLifeSig_cnt : Inport  Port=556
  VPMM_V2BAux1OnOff_enum : Inport  Port=557
  VPMM_V2BAux2OnOff_enum : Inport  Port=558
  VPMM_V2BAux3OnOff_enum : Inport  Port=559
  VPMM_V2BMainPosRlySta_enum : Inport  Port=560
  VPMM_V2BMainPosRlyFit_enum : Inport  Port=561
  VPMM_V2BACPosRlySta_enum : Inport  Port=562
  VPMM_V2BACPosRlyFit_enum : Inport  Port=563
  VPMM_V2BAirPosRlySta_enum : Inport  Port=564
  VPMM_V2BAirPosRlyFit_enum : Inport  Port=565
  VPMM_V2BOilPosRlySta_enum : Inport  Port=566
  VPMM_V2BOilPosRlyFit_enum : Inport  Port=567
  VPMM_V2BDCDCPosRlySta_enum : Inport  Port=568
  VPMM_V2BDCDCPosRlyFit_enum : Inport  Port=569
  VPMM_V2BAux1RlySta_enum : Inport  Port=570
  VPMM_V2BAux1RlyFit_enum : Inport  Port=571
  VPMM_V2BAux2RlySta_enum : Inport  Port=572
  VPMM_V2BAux2RlyFit_enum : Inport  Port=573
  VPMM_V2BAux3RlySta_enum : Inport  Port=574
  VPMM_V2BAux3RlyFit_enum : Inport  Port=575
  VPMM_V2BAux4RlySta_enum : Inport  Port=576
  VPMM_V2BAux4RlyFit_enum : Inport  Port=577
  VPMM_VCULife1_cnt : Inport  Port=578
  VPMM_VCULife2_cnt : Inport  Port=579
  VPMM_VSPFunc_enum : Inport  Port=580
  VPMM_VSPIGNKeySta_enum : Inport  Port=581
  VPMM_VSPReversed_flg : Inport  Port=582
  VPMM_VSPTurnRight_enum : Inport  Port=583
  VPMM_VSPTurnLeft_enum : Inport  Port=584
  VPMM_FogTMSRlyCMD_enum : Inport  Port=585
  VPMM_DCCurr_A : Inport  Port=586
  VPMM_DCVol_V : Inport  Port=587
  VPSA_Keystatus_enum : Inport  Port=588
  VPSA_EmergencyShutDown_flg : Inport  Port=589
  VSCP_triggerBAM_flg : Inport  Port=590
  VSCP_CFGEM1Ctrl_raw : Inport  Port=591
  VSCP_CFGEM1BAMTSize_raw : Inport  Port=592
  VSCP_CFGEM1BAMTNum_raw : Inport  Port=593
  VSCP_CFGEM1BAMRsv_raw : Inport  Port=594
  VSCP_CFGEM1BAMPGN_raw : Inport  Port=595
  VSCP_triggerDT_flg : Inport  Port=596
  VSCP_DTbyte0_raw : Inport  Port=597
  VSCP_DTbyte1_raw : Inport  Port=598
  VSCP_DTbyte2_raw : Inport  Port=599
  VSCP_DTbyte3_raw : Inport  Port=600
  VSCP_DTbyte4_raw : Inport  Port=601
  VSCP_DTbyte5_raw : Inport  Port=602
  VSCP_DTbyte6_raw : Inport  Port=603
  VSCP_DTbyte7_raw : Inport  Port=604
  VSYS_HWVer1_cnt : Inport  Port=605
  VSYS_HWVer2_cnt : Inport  Port=606
  VSYS_HWVer3_cnt : Inport  Port=607
  VSYS_CarModel1_cnt : Inport  Port=608
  VSYS_CarModel2_cnt : Inport  Port=609
  VSYS_CarModel3_cnt : Inport  Port=610
  VSYS_ECU1_cnt : Inport  Port=611
  VSYS_ECU2_cnt : Inport  Port=612
  VSYS_Major1_cnt : Inport  Port=613
  VSYS_Major2_cnt : Inport  Port=614
  VSYS_Minor1_cnt : Inport  Port=615
  VSYS_Minor2_cnt : Inport  Port=616
  VSYS_Patch1_cnt : Inport  Port=617
  VSYS_Patch2_cnt : Inport  Port=618
  VSYS_Country1_cnt : Inport  Port=619
  VSYS_Country2_cnt : Inport  Port=620
  VSYS_Variation_cnt : Inport  Port=621
  VSYS_Dash1_cnt : Inport  Port=622
  VSYS_Change1_cnt : Inport  Port=623
  VSYS_Change2_cnt : Inport  Port=624
  VSYS_Dash2_cnt : Inport  Port=625
  VSYS_SHA1_cnt : Inport  Port=626
  VSYS_SHA2_cnt : Inport  Port=627
  VSYS_SHA3_cnt : Inport  Port=628
  VSYS_SHA4_cnt : Inport  Port=629
  VSYS_SHA5_cnt : Inport  Port=630
  VSYS_SHA6_cnt : Inport  Port=631
  VSYS_SHA7_cnt : Inport  Port=632
  VSYS_SHA8_cnt : Inport  Port=633
  VSYS_NvWriteReqRisingEdge_flg : Inport  Port=634
  VSYS_FdcSlpReqRisingEdge_flg : Inport  Port=635
  VSYS_FdcSlpTime_sec : Inport  Port=636
  VSYS_PmicBootReason_enum : Inport  Port=637
  VSYS_WisrBootReason_raw32 : Inport  Port=638
  VSYS_AcoreRebootCmdACK_flg : Inport  Port=639
  VSYS_CurrentNmState_enum : Inport  Port=640
  VSYS_ECUGen1_cnt : Inport  Port=641
  VSYS_ECUGen2_cnt : Inport  Port=642
  VSYS_PmicBootPath_raw32 : Inport  Port=643
  VSYS_DrivingMode_cnt : Inport  Port=644
  VSYS_ModelYear_cnt : Inport  Port=645
  VTHC_EWPPEReq_rpm : Inport  Port=646
  VTHC_CoolFanReq_pct : Inport  Port=647
  VTHC_AfterrunningMode_flg : Inport  Port=648
  VTPM_LFBatWarn_flg : Inport  Port=649
  VTPM_RFBatWarn_flg : Inport  Port=650
  VTPM_LRBatWarn_flg : Inport  Port=651
  VTPM_RRBatWarn_flg : Inport  Port=652
  VTPM_LFWheelPress_raw8 : Inport  Port=653
  VTPM_RFWheelPress_raw8 : Inport  Port=654
  VTPM_LRWheelPress_raw8 : Inport  Port=655
  VTPM_RRWheelPress_raw8 : Inport  Port=656
  VTPM_LFWheelTemp_C : Inport  Port=657
  VTPM_RFWheelTemp_C : Inport  Port=658
  VTPM_LRWheelTemp_C : Inport  Port=659
  VTPM_RRWheelTemp_C : Inport  Port=660
  VTPM_LFSensorFail_flg : Inport  Port=661
  VTPM_RFSensorFail_flg : Inport  Port=662
  VTPM_LRSensorFail_flg : Inport  Port=663
  VTPM_RRSensorFail_flg : Inport  Port=664
  VTPM_LFWheelDebug_flg : Inport  Port=665
  VTPM_LRWheelDebug_flg : Inport  Port=666
  VTPM_RFWheelDebug_flg : Inport  Port=667
  VTPM_RRWheelDebug_flg : Inport  Port=668
  VTPM_TPMSResButtAllow_flg : Inport  Port=669
  VTPM_TPMSCaliButtAllow_flg : Inport  Port=670
  VTPM_LFPressIndi_enum : Inport  Port=671
  VTPM_RFPressIndi_enum : Inport  Port=672
  VTPM_LRPressIndi_enum : Inport  Port=673
  VTPM_RRPressIndi_enum : Inport  Port=674
  VTPM_TPMSWarnIndi_enum : Inport  Port=675
  VTPM_LFWheelTmpIndi_flg : Inport  Port=676
  VTPM_RFWheelTmpIndi_flg : Inport  Port=677
  VTPM_LRWheelTmpIndi_flg : Inport  Port=678
  VTPM_RRWheelTmpIndi_flg : Inport  Port=679
  VTPM_LFWheelPSW_raw8 : Inport  Port=680
  VTPM_LRWheelPSW_raw8 : Inport  Port=681
  VTPM_RFWheelPSW_raw8 : Inport  Port=682
  VTPM_RRWheelPSW_raw8 : Inport  Port=683
  VTPM_CWheelTips_enum : Inport  Port=684
  VTPM_AutoLTips_enum : Inport  Port=685
  VTPM_LFSensorMode_flg : Inport  Port=686
  VTPM_RFSensorMode_flg : Inport  Port=687
  VTPM_LRSensorMode_flg : Inport  Port=688
  VTPM_RRSensorMode_flg : Inport  Port=689
  VTPM_S1ID_raw32 : Inport  Port=690
  VTPM_S2ID_raw32 : Inport  Port=691
  VTPM_S3ID_raw32 : Inport  Port=692
  VTPM_S4ID_raw32 : Inport  Port=693
  VTPM_S1L_enum : Inport  Port=694
  VTPM_S2L_enum : Inport  Port=695
  VTPM_S3L_enum : Inport  Port=696
  VTPM_S4L_enum : Inport  Port=697
  VTPM_ALFin_flg : Inport  Port=698
  VTPM_LFP20_raw8 : Inport  Port=699
  VTPM_RFP20_raw8 : Inport  Port=700
  VTPM_LRP20_raw8 : Inport  Port=701
  VTPM_RRP20_raw8 : Inport  Port=702
  VTPM_FAT_flg : Inport  Port=703
  VTPM_IDin_raw32 : Inport  Port=704
  VTPM_S1WheelDebugALTU_pct : Inport  Port=705
  VTPM_S2WheelDebugALTU_pct : Inport  Port=706
  VTPM_S3WheelDebugALTU_pct : Inport  Port=707
  VTPM_S4WheelDebugALTU_pct : Inport  Port=708
  VTPM_ID1messageALTU_raw8 : Inport  Port=709
  VTPM_ID2messageALTU_raw8 : Inport  Port=710
  VTPM_ID3messageALTU_raw8 : Inport  Port=711
  VTPM_ID4messageALTU_raw8 : Inport  Port=712
  VTPM_Chkfin_flg : Inport  Port=713
  VTPM_SetIDLoc_flg : Inport  Port=714
  VTPM_TPMSStorge_flg : Inport  Port=715
  VTPM_ChkStorge_flg : Inport  Port=716
  VTPM_TPMSResButt_flg : Inport  Port=717
  VTPM_LFPindi_enum : Inport  Port=718
  VTPM_RFPind_enum : Inport  Port=719
  VTPM_LRPindi_enum : Inport  Port=720
  VTPM_RRPindi_enum : Inport  Port=721
  VTPM_WriteChkLFID_raw : Inport  Port=722
  VTPM_WriteChkRFID_raw : Inport  Port=723
  VTPM_WriteChkLRID_raw : Inport  Port=724
  VTPM_WriteChkRRID_raw : Inport  Port=725
  VTPM_WriteChkfinLFID_raw : Inport  Port=726
  VTPM_WriteChkfinRFID_raw : Inport  Port=727
  VTPM_WriteChkfinLRID_raw : Inport  Port=728
  VTPM_WriteChkfinRRID_raw : Inport  Port=729
  VTPM_Flashchkdatavalid_enum : Inport  Port=730
  VTPM_Flashdatavalid_enum : Inport  Port=731
  VTPM_unlearnSfali_flg : Inport  Port=732
  VTPM_unlearnSfailvalid_enum : Inport  Port=733
  VTPM_Prepresstempvalid_enum : Inport  Port=734
  VTPM_FlashS1ID_raw : Inport  Port=735
  VTPM_FlashS2ID_raw : Inport  Port=736
  VTPM_FlashS3ID_raw : Inport  Port=737
  VTPM_FlashS4ID_raw : Inport  Port=738
  VTPM_FlashIDvalid_enum : Inport  Port=739
  VTPM_WritingCnt_enum : Inport  Port=740
  VTPM_TPMSTLCmd_flg : Inport  Port=741
  VTPM_LProgress_enum : Inport  Port=742
  VTPM_TPMSSensorIDRegStart_flg : Inport  Port=743
  VTPM_ModelVersion_raw : Inport  Port=744
  VTPM_ModelVersionChksum_raw : Inport  Port=745
  VTQD_VCUMCUCtrlMdTQD_enum : Inport  Port=746
  VTQD_CreepSpdReq_rpm : Inport  Port=747
  VTQD_CreepIND_enum : Inport  Port=748
  VTQD_ActTUpAIND_enum : Inport  Port=749
  VTQD_VCUMCUDemHiPosVal_rpm : Inport  Port=750
  VTQD_VehAcclLimitTG_mps2 : Inport  Port=751
  VTQD_VCUEBSHHSw_enum : Inport  Port=752
  VTQD_VCUEBSRd4BR_enum : Inport  Port=753
  VTQD_ParkingProtectWarning_flg : Inport  Port=754
  VTQD_ActDriveMode_enum : Inport  Port=755
  VTQD_VCU4PweLmtInd_flg : Inport  Port=756
  VTQD_GearFlashIndDis_flg : Inport  Port=757
  VTQD_GearFlashInd_flg : Inport  Port=758
  VTQD_SpdLimSta_flg : Inport  Port=759
  VTQD_VehSpdLimitTG_kph : Inport  Port=760
  VTQD_VCUTMVehSpd_kph : Inport  Port=761
  VTQD_TMTqReq_Nm : Inport  Port=762
  VTQD_VCUBCMBuzzReq_flg : Inport  Port=763
  VTQD_VCUEBSHBSw_enum : Inport  Port=764
  VTQD_EVCU1ActDrvMode_enum : Inport  Port=765
  VTQD_EVCU1WheelSlipdet_enum : Inport  Port=766
  VTQD_EVCU1EMotorSpd_rpm : Inport  Port=767
  VTQD_EVCU1EMotorOvrerSpd_enum : Inport  Port=768
  VTQD_EVCU1EMotorPerformance_pct : Inport  Port=769
  VTQD_EVCU1EBrakeTorqLow_enum : Inport  Port=770
  VTQD_EVCU2MaxTorqAvail_pct : Inport  Port=771
  VTQD_EVCU2MinTorqAvail_pct : Inport  Port=772
  VTQD_EEC3NFricPercTorq_pct : Inport  Port=773
  VTQD_EEC3EMPressLoss_pct : Inport  Port=774
  VTQD_ETC2ActDriveDirect_enum : Inport  Port=775
  VTQD_RC1PctTrqP4_pct : Inport  Port=776
  VTQD_RC1PctTrqPekTrqP5_pct : Inport  Port=777
  VTQD_EMRC1EMTquModeDrvBrk_enum : Inport  Port=778
  VTQD_EMRC1ActEMpTrq_pct : Inport  Port=779
  VTQD_EMRC1ActEMOutSftSpd_rpm : Inport  Port=780
  VTQD_EMRC1ActEMpTrqHrls_pct : Inport  Port=781
  VTQD_EMRC1ActMaxAvaEMRecpTrq_pct : Inport  Port=782
  VTQD_EC1EMSpdIdleP1_rpm : Inport  Port=783
  VTQD_EC1PercTorqIdleP1_pct : Inport  Port=784
  VTQD_EC1EMSpdIdleP2_rpm : Inport  Port=785
  VTQD_EC1PercTorqIdleP2_pct : Inport  Port=786
  VTQD_EC1EMSpdIdleP3_rpm : Inport  Port=787
  VTQD_EC1PercTorqIdleP3_pct : Inport  Port=788
  VTQD_EC1EMSpdIdleP4_rpm : Inport  Port=789
  VTQD_EC1PercTorqIdleP4_pct : Inport  Port=790
  VTQD_EC1PercTorqIdleP5_pct : Inport  Port=791
  VTQD_EC1EMSpdIdleP5_rpm : Inport  Port=792
  VTQD_EC1EMRefTorq_Nm : Inport  Port=793
  VTQD_EC1EMMaxMEngOvrSP7_rpm : Inport  Port=794
  VTQD_EC1EMMaxMOvrTmt_s : Inport  Port=795
  VTQD_EC1EMReqSpdCtrlLoLmt_rpm : Inport  Port=796
  VTQD_EC1EMReqTrqCtrlLoLmt_pct : Inport  Port=797
  VTQD_EC1EMReqSpdCtrlUpLmt_rpm : Inport  Port=798
  VTQD_EC1EMReqTrqCtrlUpLmt_pct : Inport  Port=799
  VTQD_EC1EMExtRSCtrlUpLmt_rpm : Inport  Port=800
  VTQD_EC1EMMomOfInertia_kgpm2 : Inport  Port=801
  VTQD_EC1EMDefTrqLmt_rpm : Inport  Port=802
  VTQD_EC1EMSupVarRTSC1MSG_cnt : Inport  Port=803
  VTQD_EC1EMSupTSC1CtrlPG1_cnt : Inport  Port=804
  VTQD_EC1EMSupTSC1CtrlPG3_cnt : Inport  Port=805
  VTQD_EC1EMSupTSC1CtrlPG2_cnt : Inport  Port=806
  VTQD_EC1EMSupTSC1CtrlPG4_cnt : Inport  Port=807
  VTQD_EC1EMSpdHdleP6_rpm : Inport  Port=808
  VTQD_EC1EMGainEndSpdGvn_gain : Inport  Port=809
  VTQD_RC1RetType_enum : Inport  Port=810
  VTQD_RC1RetLocat_enum : Inport  Port=811
  VTQD_RC1RetCtrlMth_enum : Inport  Port=812
  VTQD_RC1RetSpdIdleP1_rpm : Inport  Port=813
  VTQD_RC1PctTrqIdleP1_pct : Inport  Port=814
  VTQD_RC1MaxRetSpdP2_rpm : Inport  Port=815
  VTQD_RC1RetSpdP2_pct : Inport  Port=816
  VTQD_RC1MaxRetSpdP3_rpm : Inport  Port=817
  VTQD_RC1PctTrqP3_pct : Inport  Port=818
  VTQD_RC1RefRetTrq_Nm : Inport  Port=819
  VTQD_RC1RetSpdPekTrqP5_Nm : Inport  Port=820
  VTQD_RC1RetSpdP4_rpm : Inport  Port=821
  VTQD_VCUMCUDemLoNegVal_rpm : Inport  Port=822
  VTQD_VCUMCUDemSpd_rpm : Inport  Port=823
  VTQD_VCUMCUGearSta_enum : Inport  Port=824
  VTQD_TUpAIND_enum : Inport  Port=825
  VTQD_ETC1ShiftrPgs_enum : Inport  Port=826
  VTQD_EVCU1RecuperHighSta_enum : Inport  Port=827
  VTQD_EMRC1DrvDemEMRtapTrq_pct : Inport  Port=828
  VTQD_EMRC1RetSelNonEng_pct : Inport  Port=829
  VTQD_EMRC1SACtrlDev_cnt : Inport  Port=830
  VTQD_VCUMCUHandBrk_flg : Inport  Port=831
  VTQD_VCUMCUFootBrk_flg : Inport  Port=832
  VTQR_FrTMTqReq_Nm : Inport  Port=833
  VTQR_RrTMTqReq_Nm : Inport  Port=834
  VV2L_ReqOBCV2LEna_enum : Inport  Port=835
  VV2L_ReqV2LIVIPopup_enum : Inport  Port=836
  VV2L_ReqV2LIVIDisChrg_enum : Inport  Port=837
  VV2L_ReqOBCExtrV2LEna_enum : Inport  Port=838
  VV2L_ReqOBCIntrV2LEna_enum : Inport  Port=839
  VV2L_HVPO120VGrpALDSt_enum : Inport  Port=840
  VV2L_HVPO120VGrpBLDSt_enum : Inport  Port=841
  VVMC_FeatSetSpdFinal_raw32 : Inport  Port=842
  VVMC_VehicleSpeed_mph : Inport  Port=843
  VVMC_VehicleSpeed_kph : Inport  Port=844
  VVMC_MeterIndSpeed_raw32 : Inport  Port=845
  VVMC_VMCAEBCtrlAvail_flg : Inport  Port=846
  VVMC_VMCACCCtrlAvail_flg : Inport  Port=847
  VVMC_VMCCCCtrlAvail_flg : Inport  Port=848
  VVMC_VMCMSACtrlAvail_flg : Inport  Port=849
  VVMC_FeatArbitrSta_enum : Inport  Port=850
  VVMC_FeatReqSpd_kph : Inport  Port=851
  VVMC_JerkPCT_pct : Inport  Port=852
  VVMC_LimitPCT_pct : Inport  Port=853
  VVMC_FrontRearSlipRatioCtrl_flg : Inport  Port=854
  VVMC_RearWhlSlipRatioCtrl_flg : Inport  Port=855
  VVMC_SingleWhlSlipRatioCtrl_flg : Inport  Port=856
  VVMC_LatAccCtrl_flg : Inport  Port=857
  VVMC_SafetyCtrl_flg : Inport  Port=858
  VVMC_SPD2ACCAct_flg : Inport  Port=859
  VVMC_AccCalcuPID_mps2 : Inport  Port=860
  VVMC_ISOAccLimit_mps2 : Inport  Port=861
  VVMC_ISODecLimit_mps2 : Inport  Port=862
  VVMC_ISOJerkLimit_mps3 : Inport  Port=863
  VVMC_ACCRequiredAccel_mps2 : Inport  Port=864
  VVMC_DISCReqAcc_mps2 : Inport  Port=865
  VVMC_FeatArbitrFinal_enum : Inport  Port=866
  VVMC_ActACCRequiredAccel_mps2 : Inport  Port=867
  VVMC_LateralCtrl_flg : Inport  Port=868
  VVMC_ADASLKASta_enum : Inport  Port=869
  VVMC_LKAStrToqReq_Nm : Inport  Port=870
  VVMC_LKATOIFault_flg : Inport  Port=871
  VVMC_LKATOIAct_enum : Inport  Port=872
  VVMC_ADASAEBReq_enum : Inport  Port=873
  VVMC_ADASFaultSta_flg : Inport  Port=874
  VVMC_AEBVehHoldReq_flg : Inport  Port=875
  VVMC_ACCVehHoldReq_flg : Inport  Port=876
  VVMC_ADASDBSReq_enum : Inport  Port=877
  VVMC_ADASACCSta_enum : Inport  Port=878
  VVMC_ACCObjDist_m : Inport  Port=879
  VVMC_ACCObjRelSpd_mps : Inport  Port=880
  VVMC_TimeGapLevel_enum : Inport  Port=881
  VVMC_ACCJerkUpperLimit_mps3 : Inport  Port=882
  VVMC_ACCComfortBandUpper_mps2 : Inport  Port=883
  VVMC_ACCJerkLowerLimit_mps3 : Inport  Port=884
  VVMC_ACCComfortBandLower_mps2 : Inport  Port=885
  VVMC_ADASVehSpdLim_raw32 : Inport  Port=886
  VVMC_ADASShftPosnReqA_flg : Inport  Port=887
  VVMC_ADASShftPosnReq_enum : Inport  Port=888
  VVMC_ADASForceIdle_flg : Inport  Port=889
  VVMC_HazardWarningReq_flg : Inport  Port=890
  VVMC_RightTurnLightReq_flg : Inport  Port=891
  VVMC_LeftTurnLightReq_flg : Inport  Port=892
  VVMC_ADASFCWSta_enum : Inport  Port=893
  VVMC_ADASLDWSta_enum : Inport  Port=894
  VVMC_ADASFltWrnReq_flg : Inport  Port=895
  VVMC_ACCObjDstLvl_enum : Inport  Port=896
  VVMC_ForceLowBeam_enum : Inport  Port=897
  VVMC_ACCTakeoverReq_flg : Inport  Port=898
  VVMC_ADASWarningMsg_enum : Inport  Port=899
  VVMC_ADASCAMSpdLim_enum : Inport  Port=900
  VVMC_TargetType_enum : Inport  Port=901
  VVMC_ADASSLIFSpdLim_enum : Inport  Port=902
  VVMC_LKAHODDisplayWarning_flg : Inport  Port=903
  VVMC_LKAHODSoundWarning_flg : Inport  Port=904
  VVMC_ADASLFCSta_enum : Inport  Port=905
  VVMC_ADASLaneModeL_enum : Inport  Port=906
  VVMC_ADASLaneModeR_enum : Inport  Port=907
  VVMC_ADASSLIFSta_enum : Inport  Port=908
  VVMC_ADASISASta_enum : Inport  Port=909
  VVMC_ADASLDWMute_flg : Inport  Port=910
  VVMC_ADASFCWMute_flg : Inport  Port=911
  VVMC_ADASLFCHandsOffWarning_enum : Inport  Port=912
  VVMC_LVDADisabled_flg : Inport  Port=913
  VVMC_LVDAMuteSta_enum : Inport  Port=914
  VVMC_LVDAFailinfo_flg : Inport  Port=915
  VVMC_LVDAWarning_flg : Inport  Port=916
  VVMC_LVDAACCStatusInformation_flg : Inport  Port=917
  VVMC_ADASLFCWarnSound_enum : Inport  Port=918
  VVMC_FCMACCmode_enum : Inport  Port=919
  VVMC_ADASLanetypeR_enum : Inport  Port=920
  VVMC_ADASLanetypeL_enum : Inport  Port=921
  VVMC_ADASLanecurveL_raw32 : Inport  Port=922
  VVMC_ADASLanecurveR_raw32 : Inport  Port=923
  VVMC_ADASAEBSta_enum : Inport  Port=924
  VVMC_FCMLDWRequest_enum : Inport  Port=925
  VVMC_FCMLDWFault_flg : Inport  Port=926
  VVMC_ACCCtrlAvail_flg : Inport  Port=927
  VVMC_ACCPedalOvrd_flg : Inport  Port=928
  VVMC_TimeGapCalcu_s : Inport  Port=929
  VVMC_CCCtrlSta_enum : Inport  Port=930
  VVMC_MSACtrlSta_enum : Inport  Port=931
  VVMC_APSCtrlAvail_flg : Inport  Port=932
  VVMC_APSActive_flg : Inport  Port=933
  VVMC_APSStaSys_enum : Inport  Port=934
  VVMC_APSDecReqA_flg : Inport  Port=935
  VVMC_APSDecReq_mps2 : Inport  Port=936
  VVMC_APSReq_enum : Inport  Port=937
  VVMC_LongAcc_Gps : Inport  Port=938
  VVMC_CCMSASpdWar_flg : Inport  Port=939
  VVMC_IMUEnaCmd_flg : Inport  Port=940
  VVMC_CAASCtrlAvail_flg : Inport  Port=941
  VVMC_CAASActive_flg : Inport  Port=942
  VVMC_ExtraMSACtrlSta_enum : Inport  Port=943
  VVMC_CalibratedAccX_G : Inport  Port=944
  VVMC_CalibratedAccY_G : Inport  Port=945
  VVMC_CalibratedAccZ_G : Inport  Port=946
  VVMC_CalibratedGyroX_Dps : Inport  Port=947
  VVMC_CalibratedGyroY_Dps : Inport  Port=948
  VVMC_CalibratedGyroZ_Dps : Inport  Port=949
  VVMC_FDCVMCAPSVRqEPSCtrl_flg : Inport  Port=950
  VVMC_FDCVMCAPSAngleTarget_deg : Inport  Port=951
  VVMC_FDCVMCAPSRqEPSCtrl_flg : Inport  Port=952
  VVMC_FDCVMCAngCtrlTqWtGn_pct : Inport  Port=953
  VVMC_FDCVMCDrInpTqBstAct_flg : Inport  Port=954
  VVMC_FDCVMCMaxAngCtrlOutTqLim_Nm : Inport  Port=955
  VVMC_FDCVMCDrInpTqBstGn_pct : Inport  Port=956
  UnitConverter{1,5,13,18,20..28,33..40,53..54,56,75,77,79,81,91,93,95,97,99,101,103,139,145,147,149,151,153,159,161,170..173,177..179,182,185,187..188,213,223,227..232,234,294,379,388,405,473..478,488..490,492..493,495,498..510,515,519,521..522,525,527,529..535,538..546,551,556..581,583..585,588,591,593..594,597..633,637,640..642,644..645,653..656,671..675,680..685,694..697,699..702,709..712,718..721,730..731,733..734,739..740,742,744..746,748..749,752..753,755,764..766,768,770,778,803..807,810..811,824..827,830,835..841,850,866,869,872..873,877..878,881,888,893..894,896..897,899..902,905..909,912,914,918..921,924..925,930..931,934,937,943} (297 alike) : DataTypeConversion  OutDataTypeStr=uint8
  UnitConverter{2..4,6..8,10..12,17,19,41..52,55,58,60,62,64,66..74,76,78,80,82..90,92,94,96,98,100,102,104,106,108..114,116,118,120,122,124..138,140..144,146,148,150,152,154..158,160,162..168,175..176,180..181,184,186,189..212,214..222,224..226,233,235..246,293,304,378,380..387,389..395,399,497,511..513,516..518,520,523..524,526,528,536..537,547..550,552..555,582,589..590,596,634..635,639,648..652,661..670,676..679,686..689,698,703,713..717,732,741,743,754,756..759,763,831..832,846..849,854..859,868,871,874..876,887,889..892,895,898,903..904,910..911,913,915..917,926..928,932..933,935,939..942,950,952,954} (292 alike) : DataTypeConversion  OutDataTypeStr=boolean
  UnitConverter{9,14..16,57,59,61,63,65,105,107,115,117,119,121,123,169,174,183,396..398,400..402,404,406..408,411..419,421,428..429,431..455,460..463,470..472,479..480,491,514,586..587,636,646..647,657..660,705..708,747,750..751,760..762,767,769,771..777,779..802,808..809,812..823,828..829,833..834,842..845,851..853,860..865,867,870,879..880,882..886,922..923,929,936,938,944..949,951,953,955..956} (184 alike) : DataTypeConversion  OutDataTypeStr=single
  UnitConverter{247..292,295..303,305..377,422..427,456..457,464..469,481..487,494,496,595,638,643,690..693,704,722..729,735..738} (171 alike) : DataTypeConversion  OutDataTypeStr=uint32
  UnitConverter{29..32,403,409..410,420,430,458..459,592} (12 alike) : DataTypeConversion  OutDataTypeStr=uint16
  VACC_CACFanReq_flg_Inproc : FVT_lib/outp/OverrideAndLimit  SystemSampleTime=-1  VariantActivationTime=update diagram  Latency=0  AutoFrameSizeCalculation=off
      link override Signal_Limit/_maxval: Value=KOUTP_CACFanReq_flg_maxval
      link override Signal_Limit/_minval: Value=KOUTP_CACFanReq_flg_minval
      link override Signal_Override/_ovrdflg: Value=KOUTP_CACFanReq_flg_ovrdflg
      link override Signal_Override/_ovrdval: Value=KOUTP_CACFanReq_flg_ovrdval
  VACC_CACOverrun_flg_Inproc : FVT_lib/outp/OverrideAndLimit  SystemSampleTime=-1  VariantActivationTime=update diagram  Latency=0  AutoFrameSizeCalculation=off
      link override Signal_Limit/_maxval: Value=KOUTP_CACOverrun_flg_maxval
      link override Signal_Limit/_minval: Value=KOUTP_CACOverrun_flg_minval
      link override Signal_Override/_ovrdflg: Value=KOUTP_CACOverrun_flg_ovrdflg
      link override Signal_Override/_ovrdval: Value=KOUTP_CACOverrun_flg_ovrdval
  VACC_CACPresReady_flg_Inproc : FVT_lib/outp/OverrideAndLimit  SystemSampleTime=-1  VariantActivationTime=update diagram  Latency=0  AutoFrameSizeCalculation=off
      link override Signal_Limit/_maxval: Value=KOUTP_CACPresReady_flg_maxval
      link override Signal_Limit/_minval: Value=KOUTP_CACPresReady_flg_minval
      link override Signal_Override/_ovrdflg: Value=KOUTP_CACPresReady_flg_ovrdflg
      link override Signal_Override/_ovrdval: Value=KOUTP_CACPresReady_flg_ovrdval
  VACC_CACPresWarn_flg_Inproc : FVT_lib/outp/OverrideAndLimit  SystemSampleTime=-1  VariantActivationTime=update diagram  Latency=0  AutoFrameSizeCalculation=off
      link override Signal_Limit/_maxval: Value=KOUTP_CACPresWarn_flg_maxval
      link override Signal_Limit/_minval: Value=KOUTP_CACPresWarn_flg_minval
      link override Signal_Override/_ovrdflg: Value=KOUTP_CACPresWarn_flg_ovrdflg
      link override Signal_Override/_ovrdval: Value=KOUTP_CACPresWarn_flg_ovrdval
  VACC_CACRunFail_flg_Inproc : FVT_lib/outp/OverrideAndLimit  SystemSampleTime=-1  VariantActivationTime=update diagram  Latency=0  AutoFrameSizeCalculation=off
      link override Signal_Limit/_maxval: Value=KOUTP_CACRunFail_flg_maxval
      link override Signal_Limit/_minval: Value=KOUTP_CACRunFail_flg_minval
      link override Signal_Override/_ovrdflg: Value=KOUTP_CACRunFail_flg_ovrdflg
      link override Signal_Override/_ovrdval: Value=KOUTP_CACRunFail_flg_ovrdval
  VACC_CACTempOverHigh_flg_Inproc : FVT_lib/outp/OverrideAndLimit  SystemSampleTime=-1  VariantActivationTime=update diagram  Latency=0  AutoFrameSizeCalculation=off
      link override Signal_Limit/_maxval: Value=KOUTP_CACTempOverHigh_flg_maxval
      link override Signal_Limit/_minval: Value=KOUTP_CACTempOverHigh_flg_minval
      link override Signal_Override/_ovrdflg: Value=KOUTP_CACTempOverHigh_flg_ovrdflg
      link override Signal_Override/_ovrdval: Value=KOUTP_CACTempOverHigh_flg_ovrdval
  VACC_DCDCEnDemamd_enum_Inproc : FVT_lib/outp/OverrideAndLimit  SystemSampleTime=-1  VariantActivationTime=update diagram  Latency=0  AutoFrameSizeCalculation=off
      link override Signal_Limit/_maxval: Value=KOUTP_DCDCEnDemamd_enum_maxval
      link override Signal_Limit/_minval: Value=KOUTP_DCDCEnDemamd_enum_minval
      link override Signal_Override/_ovrdflg: Value=KOUTP_DCDCEnDemamd_enum_ovrdflg
      link override Signal_Override/_ovrdval: Value=KOUTP_DCDCEnDemamd_enum_ovrdval
  VACC_EACEnDemand_enum_Inproc : FVT_lib/outp/OverrideAndLimit  SystemSampleTime=-1  VariantActivationTime=update diagram  Latency=0  AutoFrameSizeCalculation=off
      link override Signal_Limit/_maxval: Value=KOUTP_EACEnDemand_enum_maxval
      link override Signal_Limit/_minval: Value=KOUTP_EACEnDemand_enum_minval
      link override Signal_Override/_ovrdflg: Value=KOUTP_EACEnDemand_enum_ovrdflg
      link override Signal_Override/_ovrdval: Value=KOUTP_EACEnDemand_enum_ovrdval
  VACC_EACSpdDemand_rpm_Inproc : FVT_lib/outp/OverrideAndLimit  SystemSampleTime=-1  VariantActivationTime=update diagram  Latency=0  AutoFrameSizeCalculation=off
      link override Signal_Limit/_maxval: Value=KOUTP_EACSpdDemand_rpm_maxval
      link override Signal_Limit/_minval: Value=KOUTP_EACSpdDemand_rpm_minval
      link override Signal_Override/_ovrdflg: Value=KOUTP_EACSpdDemand_rpm_ovrdflg
      link override Signal_Override/_ovrdval: Value=KOUTP_EACSpdDemand_rpm_ovrdval
  VACC_EHPSDisEnTimeout_flg_Inproc : FVT_lib/outp/OverrideAndLimit  SystemSampleTime=-1  VariantActivationTime=update diagram  Latency=0  AutoFrameSizeCalculation=off
      link override Signal_Limit/_maxval: Value=KOUTP_EHPSDisEnTimeout_flg_maxval
      link override Signal_Limit/_minval: Value=KOUTP_EHPSDisEnTimeout_flg_minval
      link override Signal_Override/_ovrdflg: Value=KOUTP_EHPSDisEnTimeout_flg_ovrdflg
      link override Signal_Override/_ovrdval: Value=KOUTP_EHPSDisEnTimeout_flg_ovrdval
  VACC_EHPSEnDemand_enum_Inproc : FVT_lib/outp/OverrideAndLimit  SystemSampleTime=-1  VariantActivationTime=update diagram  Latency=0  AutoFrameSizeCalculation=off
      link override Signal_Limit/_maxval: Value=KOUTP_EHPSEnDemand_enum_maxval
      link override Signal_Limit/_minval: Value=KOUTP_EHPSEnDemand_enum_minval
      link override Signal_Override/_ovrdflg: Value=KOUTP_EHPSEnDemand_enum_ovrdflg
      link override Signal_Override/_ovrdval: Value=KOUTP_EHPSEnDemand_enum_ovrdval
  VACC_EHPSEnTimeout_flg_Inproc : FVT_lib/outp/OverrideAndLimit  SystemSampleTime=-1  VariantActivationTime=update diagram  Latency=0  AutoFrameSizeCalculation=off
      link override Signal_Limit/_maxval: Value=KOUTP_EHPSEnTimeout_flg_maxval
      link override Signal_Limit/_minval: Value=KOUTP_EHPSEnTimeout_flg_minval
      link override Signal_Override/_ovrdflg: Value=KOUTP_EHPSEnTimeout_flg_ovrdflg
      link override Signal_Override/_ovrdval: Value=KOUTP_EHPSEnTimeout_flg_ovrdval
  VACC_EHPSMotorDemSpd_rpm_Inproc : FVT_lib/outp/OverrideAndLimit  SystemSampleTime=-1  VariantActivationTime=update diagram  Latency=0  AutoFrameSizeCalculation=off
      link override Signal_Limit/_maxval: Value=KOUTP_EHPSMotorDemSpd_rpm_maxval
      link override Signal_Limit/_minval: Value=KOUTP_EHPSMotorDemSpd_rpm_minval
      link override Signal_Override/_ovrdflg: Value=KOUTP_EHPSMotorDemSpd_rpm_ovrdflg
      link override Signal_Override/_ovrdval: Value=KOUTP_EHPSMotorDemSpd_rpm_ovrdval
  VACC_EHPSSpdCtrlMode_enum_Inproc : FVT_lib/outp/OverrideAndLimit  SystemSampleTime=-1  VariantActivationTime=update diagram  Latency=0  AutoFrameSizeCalculation=off
      link override Signal_Limit/_maxval: Value=KOUTP_EHPSSpdCtrlMode_enum_maxval
      link override Signal_Limit/_minval: Value=KOUTP_EHPSSpdCtrlMode_enum_minval
      link override Signal_Override/_ovrdflg: Value=KOUTP_EHPSSpdCtrlMode_enum_ovrdflg
      link override Signal_Override/_ovrdval: Value=KOUTP_EHPSSpdCtrlMode_enum_ovrdval
  VACC_EHPSSpdDemTimeout_flg_Inproc : FVT_lib/outp/OverrideAndLimit  SystemSampleTime=-1  VariantActivationTime=update diagram  Latency=0  AutoFrameSizeCalculation=off
      link override Signal_Limit/_maxval: Value=KOUTP_EHPSSpdDemTimeout_flg_maxval
      link override Signal_Limit/_minval: Value=KOUTP_EHPSSpdDemTimeout_flg_minval
      link override Signal_Override/_ovrdflg: Value=KOUTP_EHPSSpdDemTimeout_flg_ovrdflg
      link override Signal_Override/_ovrdval: Value=KOUTP_EHPSSpdDemTimeout_flg_ovrdval
  VAPM_ABSActiveTimeOut_flg_Inproc : FVT_lib/outp/OverrideAndLimit  SystemSampleTime=-1  VariantActivationTime=update diagram  Latency=0  AutoFrameSizeCalculation=off
      link override Signal_Limit/_maxval: Value=KOUTP_ABSActiveTimeOut_flg_maxval
      link override Signal_Limit/_minval: Value=KOUTP_ABSActiveTimeOut_flg_minval
      link override Signal_Override/_ovrdflg: Value=KOUTP_ABSActiveTimeOut_flg_ovrdflg
      link override Signal_Override/_ovrdval: Value=KOUTP_ABSActiveTimeOut_flg_ovrdval
  VAPM_ABSActive_flg_Inproc : FVT_lib/outp/OverrideAndLimit  SystemSampleTime=-1  VariantActivationTime=update diagram  Latency=0  AutoFrameSizeCalculation=off
      link override Signal_Limit/_maxval: Value=KOUTP_ABSActive_flg_maxval
      link override Signal_Limit/_minval: Value=KOUTP_ABSActive_flg_minval
      link override Signal_Override/_ovrdflg: Value=KOUTP_ABSActive_flg_ovrdflg
      link override Signal_Override/_ovrdval: Value=KOUTP_ABSActive_flg_ovrdval
  VAPM_APSAngleTarget_Deg_Inproc : FVT_lib/outp/OverrideAndLimit  SystemSampleTime=-1  VariantActivationTime=update diagram  Latency=0  AutoFrameSizeCalculation=off
      link override Signal_Limit/_maxval: Value=KOUTP_APSAngleTarget_Deg_maxval
      link override Signal_Limit/_minval: Value=KOUTP_APSAngleTarget_Deg_minval
      link override Signal_Override/_ovrdflg: Value=KOUTP_APSAngleTarget_Deg_ovrdflg
      link override Signal_Override/_ovrdval: Value=KOUTP_APSAngleTarget_Deg_ovrdval
  VAPM_APSDFLL_cm_Inproc : FVT_lib/outp/OverrideAndLimit  SystemSampleTime=-1  VariantActivationTime=update diagram  Latency=0  AutoFrameSizeCalculation=off
      link override Signal_Limit/_maxval: Value=KOUTP_APSDFLL_cm_maxval
      link override Signal_Limit/_minval: Value=KOUTP_APSDFLL_cm_minval
      link override Signal_Override/_ovrdflg: Value=KOUTP_APSDFLL_cm_ovrdflg
      link override Signal_Override/_ovrdval: Value=KOUTP_APSDFLL_cm_ovrdval
  VAPM_APSDFLR_cm_Inproc : FVT_lib/outp/OverrideAndLimit  SystemSampleTime=-1  VariantActivationTime=update diagram  Latency=0  AutoFrameSizeCalculation=off
      link override Signal_Limit/_maxval: Value=KOUTP_APSDFLR_cm_maxval
      link override Signal_Limit/_minval: Value=KOUTP_APSDFLR_cm_minval
      link override Signal_Override/_ovrdflg: Value=KOUTP_APSDFLR_cm_ovrdflg
      link override Signal_Override/_ovrdval: Value=KOUTP_APSDFLR_cm_ovrdval
  VAPM_APSDRLL_cm_Inproc : FVT_lib/outp/OverrideAndLimit  SystemSampleTime=-1  VariantActivationTime=update diagram  Latency=0  AutoFrameSizeCalculation=off
      link override Signal_Limit/_maxval: Value=KOUTP_APSDRLL_cm_maxval
      link override Signal_Limit/_minval: Value=KOUTP_APSDRLL_cm_minval
      link override Signal_Override/_ovrdflg: Value=KOUTP_APSDRLL_cm_ovrdflg
      link override Signal_Override/_ovrdval: Value=KOUTP_APSDRLL_cm_ovrdval
  VAPM_APSDRLR_cm_Inproc : FVT_lib/outp/OverrideAndLimit  SystemSampleTime=-1  VariantActivationTime=update diagram  Latency=0  AutoFrameSizeCalculation=off
      link override Signal_Limit/_maxval: Value=KOUTP_APSDRLR_cm_maxval
      link override Signal_Limit/_minval: Value=KOUTP_APSDRLR_cm_minval
      link override Signal_Override/_ovrdflg: Value=KOUTP_APSDRLR_cm_ovrdflg
      link override Signal_Override/_ovrdval: Value=KOUTP_APSDRLR_cm_ovrdval
  VAPM_APSExitCondition_enum_Inproc : FVT_lib/outp/OverrideAndLimit  SystemSampleTime=-1  VariantActivationTime=update diagram  Latency=0  AutoFrameSizeCalculation=off
      link override Signal_Limit/_maxval: Value=KOUTP_APSExitCondition_enum_maxval
      link override Signal_Limit/_minval: Value=KOUTP_APSExitCondition_enum_minval
      link override Signal_Override/_ovrdflg: Value=KOUTP_APSExitCondition_enum_ovrdflg
      link override Signal_Override/_ovrdval: Value=KOUTP_APSExitCondition_enum_ovrdval
  VAPM_APSHWVer_enum_Inproc : FVT_lib/outp/OverrideAndLimit  SystemSampleTime=-1  VariantActivationTime=update diagram  Latency=0  AutoFrameSizeCalculation=off
      link override Signal_Limit/_maxval: Value=KOUTP_APSHWVer_enum_maxval
      link override Signal_Limit/_minval: Value=KOUTP_APSHWVer_enum_minval
      link override Signal_Override/_ovrdflg: Value=KOUTP_APSHWVer_enum_ovrdflg
      link override Signal_Override/_ovrdval: Value=KOUTP_APSHWVer_enum_ovrdval
  VAPM_APSProgressPCT_pct_Inproc : FVT_lib/outp/OverrideAndLimit  SystemSampleTime=-1  VariantActivationTime=update diagram  Latency=0  AutoFrameSizeCalculation=off
      link override Signal_Limit/_maxval: Value=KOUTP_APSProgressPCT_pct_maxval
      link override Signal_Limit/_minval: Value=KOUTP_APSProgressPCT_pct_minval
      link override Signal_Override/_ovrdflg: Value=KOUTP_APSProgressPCT_pct_ovrdflg
      link override Signal_Override/_ovrdval: Value=KOUTP_APSProgressPCT_pct_ovrdval
  VAPM_APSPwrReq_enum_Inproc : FVT_lib/outp/OverrideAndLimit  SystemSampleTime=-1  VariantActivationTime=update diagram  Latency=0  AutoFrameSizeCalculation=off
      link override Signal_Limit/_maxval: Value=KOUTP_APSPwrReq_enum_maxval
      link override Signal_Limit/_minval: Value=KOUTP_APSPwrReq_enum_minval
      link override Signal_Override/_ovrdflg: Value=KOUTP_APSPwrReq_enum_ovrdflg
      link override Signal_Override/_ovrdval: Value=KOUTP_APSPwrReq_enum_ovrdval
  VAPM_APSRQDisplay_enum_Inproc : FVT_lib/outp/OverrideAndLimit  SystemSampleTime=-1  VariantActivationTime=update diagram  Latency=0  AutoFrameSizeCalculation=off
      link override Signal_Limit/_maxval: Value=KOUTP_APSRQDisplay_enum_maxval
      link override Signal_Limit/_minval: Value=KOUTP_APSRQDisplay_enum_minval
      link override Signal_Override/_ovrdflg: Value=KOUTP_APSRQDisplay_enum_ovrdflg
      link override Signal_Override/_ovrdval: Value=KOUTP_APSRQDisplay_enum_ovrdval
  VAPM_APSRqEPASCtrl_flg_Inproc : FVT_lib/outp/OverrideAndLimit  SystemSampleTime=-1  VariantActivationTime=update diagram  Latency=0  AutoFrameSizeCalculation=off
      link override Signal_Limit/_maxval: Value=KOUTP_APSRqEPASCtrl_flg_maxval
      link override Signal_Limit/_minval: Value=KOUTP_APSRqEPASCtrl_flg_minval
      link override Signal_Override/_ovrdflg: Value=KOUTP_APSRqEPASCtrl_flg_ovrdflg
      link override Signal_Override/_ovrdval: Value=KOUTP_APSRqEPASCtrl_flg_ovrdval
  VAPM_APSSWVer_enum_Inproc : FVT_lib/outp/OverrideAndLimit  SystemSampleTime=-1  VariantActivationTime=update diagram  Latency=0  AutoFrameSizeCalculation=off
      link override Signal_Limit/_maxval: Value=KOUTP_APSSWVer_enum_maxval
      link override Signal_Limit/_minval: Value=KOUTP_APSSWVer_enum_minval
      link override Signal_Override/_ovrdflg: Value=KOUTP_APSSWVer_enum_ovrdflg
      link override Signal_Override/_ovrdval: Value=KOUTP_APSSWVer_enum_ovrdval
  VAPM_APSShiftPosnReq_enum_Inproc : FVT_lib/outp/OverrideAndLimit  SystemSampleTime=-1  VariantActivationTime=update diagram  Latency=0  AutoFrameSizeCalculation=off
      link override Signal_Limit/_maxval: Value=KOUTP_APSShiftPosnReq_enum_maxval
      link override Signal_Limit/_minval: Value=KOUTP_APSShiftPosnReq_enum_minval
      link override Signal_Override/_ovrdflg: Value=KOUTP_APSShiftPosnReq_enum_ovrdflg
      link override Signal_Override/_ovrdval: Value=KOUTP_APSShiftPosnReq_enum_ovrdval
  VAPM_APSSpeedCMD_kph_Inproc : FVT_lib/outp/OverrideAndLimit  SystemSampleTime=-1  VariantActivationTime=update diagram  Latency=0  AutoFrameSizeCalculation=off
      link override Signal_Limit/_maxval: Value=KOUTP_APSSpeedCMD_kph_maxval
      link override Signal_Limit/_minval: Value=KOUTP_APSSpeedCMD_kph_minval
      link override Signal_Override/_ovrdflg: Value=KOUTP_APSSpeedCMD_kph_ovrdflg
      link override Signal_Override/_ovrdval: Value=KOUTP_APSSpeedCMD_kph_ovrdval
  VAPM_APSVMCReqA_flg_Inproc : FVT_lib/outp/OverrideAndLimit  SystemSampleTime=-1  VariantActivationTime=update diagram  Latency=0  AutoFrameSizeCalculation=off
      link override Signal_Limit/_maxval: Value=KOUTP_APSVMCReqA_flg_maxval
      link override Signal_Limit/_minval: Value=KOUTP_APSVMCReqA_flg_minval
      link override Signal_Override/_ovrdflg: Value=KOUTP_APSVMCReqA_flg_ovrdflg
      link override Signal_Override/_ovrdval: Value=KOUTP_APSVMCReqA_flg_ovrdval
  VAPM_APSVRqEPASCtrl_flg_Inproc : FVT_lib/outp/OverrideAndLimit  SystemSampleTime=-1  VariantActivationTime=update diagram  Latency=0  AutoFrameSizeCalculation=off
      link override Signal_Limit/_maxval: Value=KOUTP_APSVRqEPASCtrl_flg_maxval
      link override Signal_Limit/_minval: Value=KOUTP_APSVRqEPASCtrl_flg_minval
      link override Signal_Override/_ovrdflg: Value=KOUTP_APSVRqEPASCtrl_flg_ovrdflg
      link override Signal_Override/_ovrdval: Value=KOUTP_APSVRqEPASCtrl_flg_ovrdval
  VAPM_AVMErrSTATimeOut_flg_Inproc : FVT_lib/outp/OverrideAndLimit  SystemSampleTime=-1  VariantActivationTime=update diagram  Latency=0  AutoFrameSizeCalculation=off
      link override Signal_Limit/_maxval: Value=KOUTP_AVMErrSTATimeOut_flg_maxval
      link override Signal_Limit/_minval: Value=KOUTP_AVMErrSTATimeOut_flg_minval
      link override Signal_Override/_ovrdflg: Value=KOUTP_AVMErrSTATimeOut_flg_ovrdflg
      link override Signal_Override/_ovrdval: Value=KOUTP_AVMErrSTATimeOut_flg_ovrdval
  VAPM_AVMErrSTA_flg_Inproc : FVT_lib/outp/OverrideAndLimit  SystemSampleTime=-1  VariantActivationTime=update diagram  Latency=0  AutoFrameSizeCalculation=off
      link override Signal_Limit/_maxval: Value=KOUTP_AVMErrSTA_flg_maxval
      link override Signal_Limit/_minval: Value=KOUTP_AVMErrSTA_flg_minval
      link override Signal_Override/_ovrdflg: Value=KOUTP_AVMErrSTA_flg_ovrdflg
      link override Signal_Override/_ovrdval: Value=KOUTP_AVMErrSTA_flg_ovrdval
  VAPM_AVMParkingmodeTimeOut_flg_Inproc : FVT_lib/outp/OverrideAndLimit  SystemSampleTime=-1  VariantActivationTime=update diagram  Latency=0  AutoFrameSizeCalculation=off
      link override Signal_Limit/_maxval: Value=KOUTP_AVMParkingmodeTimeOut_flg_maxval
      link override Signal_Limit/_minval: Value=KOUTP_AVMParkingmodeTimeOut_flg_minval
      link override Signal_Override/_ovrdflg: Value=KOUTP_AVMParkingmodeTimeOut_flg_ovrdflg
      link override Signal_Override/_ovrdval: Value=KOUTP_AVMParkingmodeTimeOut_flg_ovrdval
  VAPM_AVMParkingmode_enum_Inproc : FVT_lib/outp/OverrideAndLimit  SystemSampleTime=-1  VariantActivationTime=update diagram  Latency=0  AutoFrameSizeCalculation=off
      link override Signal_Limit/_maxval: Value=KOUTP_AVMParkingmode_enum_maxval
      link override Signal_Limit/_minval: Value=KOUTP_AVMParkingmode_enum_minval
      link override Signal_Override/_ovrdflg: Value=KOUTP_AVMParkingmode_enum_ovrdflg
      link override Signal_Override/_ovrdval: Value=KOUTP_AVMParkingmode_enum_ovrdval
  VAPM_AVMparkingcancelTimeOut_flg_Inproc : FVT_lib/outp/OverrideAndLimit  SystemSampleTime=-1  VariantActivationTime=update diagram  Latency=0  AutoFrameSizeCalculation=off
      link override Signal_Limit/_maxval: Value=KOUTP_AVMparkingcancelTimeOut_flg_maxval
      link override Signal_Limit/_minval: Value=KOUTP_AVMparkingcancelTimeOut_flg_minval
      link override Signal_Override/_ovrdflg: Value=KOUTP_AVMparkingcancelTimeOut_flg_ovrdflg
      link override Signal_Override/_ovrdval: Value=KOUTP_AVMparkingcancelTimeOut_flg_ovrdval
  VAPM_AVMparkingcancel_enum_Inproc : FVT_lib/outp/OverrideAndLimit  SystemSampleTime=-1  VariantActivationTime=update diagram  Latency=0  AutoFrameSizeCalculation=off
      link override Signal_Limit/_maxval: Value=KOUTP_AVMparkingcancel_enum_maxval
      link override Signal_Limit/_minval: Value=KOUTP_AVMparkingcancel_enum_minval
      link override Signal_Override/_ovrdflg: Value=KOUTP_AVMparkingcancel_enum_ovrdflg
      link override Signal_Override/_ovrdval: Value=KOUTP_AVMparkingcancel_enum_ovrdval
  VAPM_AVMparkingexcuteTimeOut_flg_Inproc : FVT_lib/outp/OverrideAndLimit  SystemSampleTime=-1  VariantActivationTime=update diagram  Latency=0  AutoFrameSizeCalculation=off
      link override Signal_Limit/_maxval: Value=KOUTP_AVMparkingexcuteTimeOut_flg_maxval
      link override Signal_Limit/_minval: Value=KOUTP_AVMparkingexcuteTimeOut_flg_minval
      link override Signal_Override/_ovrdflg: Value=KOUTP_AVMparkingexcuteTimeOut_flg_ovrdflg
      link override Signal_Override/_ovrdval: Value=KOUTP_AVMparkingexcuteTimeOut_flg_ovrdval
  VAPM_AVMparkingexcute_enum_Inproc : FVT_lib/outp/OverrideAndLimit  SystemSampleTime=-1  VariantActivationTime=update diagram  Latency=0  AutoFrameSizeCalculation=off
      link override Signal_Limit/_maxval: Value=KOUTP_AVMparkingexcute_enum_maxval
      link override Signal_Limit/_minval: Value=KOUTP_AVMparkingexcute_enum_minval
      link override Signal_Override/_ovrdflg: Value=KOUTP_AVMparkingexcute_enum_ovrdflg
      link override Signal_Override/_ovrdval: Value=KOUTP_AVMparkingexcute_enum_ovrdval
  VAPM_BrkPedalPosTimeOut_flg_Inproc : FVT_lib/outp/OverrideAndLimit  SystemSampleTime=-1  VariantActivationTime=update diagram  Latency=0  AutoFrameSizeCalculation=off
      link override Signal_Limit/_maxval: Value=KOUTP_BrkPedalPosTimeOut_flg_maxval
      link override Signal_Limit/_minval: Value=KOUTP_BrkPedalPosTimeOut_flg_minval
      link override Signal_Override/_ovrdflg: Value=KOUTP_BrkPedalPosTimeOut_flg_ovrdflg
      link override Signal_Override/_ovrdval: Value=KOUTP_BrkPedalPosTimeOut_flg_ovrdval
  VAPM_BrkPedalPos_pct_Inproc : FVT_lib/outp/OverrideAndLimit  SystemSampleTime=-1  VariantActivationTime=update diagram  Latency=0  AutoFrameSizeCalculation=off
      link override Signal_Limit/_maxval: Value=KOUTP_BrkPedalPos_pct_maxval
      link override Signal_Limit/_minval: Value=KOUTP_BrkPedalPos_pct_minval
      link override Signal_Override/_ovrdflg: Value=KOUTP_BrkPedalPos_pct_ovrdflg
      link override Signal_Override/_ovrdval: Value=KOUTP_BrkPedalPos_pct_ovrdval
  VAPM_BrkSwStaTimeOut_flg_Inproc : FVT_lib/outp/OverrideAndLimit  SystemSampleTime=-1  VariantActivationTime=update diagram  Latency=0  AutoFrameSizeCalculation=off
      link override Signal_Limit/_maxval: Value=KOUTP_BrkSwStaTimeOut_flg_maxval
      link override Signal_Limit/_minval: Value=KOUTP_BrkSwStaTimeOut_flg_minval
      link override Signal_Override/_ovrdflg: Value=KOUTP_BrkSwStaTimeOut_flg_ovrdflg
      link override Signal_Override/_ovrdval: Value=KOUTP_BrkSwStaTimeOut_flg_ovrdval
  VAPM_BrkSwSta_flg_Inproc : FVT_lib/outp/OverrideAndLimit  SystemSampleTime=-1  VariantActivationTime=update diagram  Latency=0  AutoFrameSizeCalculation=off
      link override Signal_Limit/_maxval: Value=KOUTP_BrkSwSta_flg_maxval
      link override Signal_Limit/_minval: Value=KOUTP_BrkSwSta_flg_minval
      link override Signal_Override/_ovrdflg: Value=KOUTP_BrkSwSta_flg_ovrdflg
      link override Signal_Override/_ovrdval: Value=KOUTP_BrkSwSta_flg_ovrdval
  VAPM_BrkSwVTimeOut_flg_Inproc : FVT_lib/outp/OverrideAndLimit  SystemSampleTime=-1  VariantActivationTime=update diagram  Latency=0  AutoFrameSizeCalculation=off
      link override Signal_Limit/_maxval: Value=KOUTP_BrkSwVTimeOut_flg_maxval
      link override Signal_Limit/_minval: Value=KOUTP_BrkSwVTimeOut_flg_minval
      link override Signal_Override/_ovrdflg: Value=KOUTP_BrkSwVTimeOut_flg_ovrdflg
      link override Signal_Override/_ovrdval: Value=KOUTP_BrkSwVTimeOut_flg_ovrdval
  VAPM_BrkSwV_flg_Inproc : FVT_lib/outp/OverrideAndLimit  SystemSampleTime=-1  VariantActivationTime=update diagram  Latency=0  AutoFrameSizeCalculation=off
      link override Signal_Limit/_maxval: Value=KOUTP_BrkSwV_flg_maxval
      link override Signal_Limit/_minval: Value=KOUTP_BrkSwV_flg_minval
      link override Signal_Override/_ovrdflg: Value=KOUTP_BrkSwV_flg_ovrdflg
      link override Signal_Override/_ovrdval: Value=KOUTP_BrkSwV_flg_ovrdval
  VAPM_CAASSta_enum_Inproc : FVT_lib/outp/OverrideAndLimit  SystemSampleTime=-1  VariantActivationTime=update diagram  Latency=0  AutoFrameSizeCalculation=off
      link override Signal_Limit/_maxval: Value=KOUTP_CAASSta_enum_maxval
      link override Signal_Limit/_minval: Value=KOUTP_CAASSta_enum_minval
      link override Signal_Override/_ovrdflg: Value=KOUTP_CAASSta_enum_ovrdflg
      link override Signal_Override/_ovrdval: Value=KOUTP_CAASSta_enum_ovrdval
  VAPM_CAASSwTimeOut_flg_Inproc : FVT_lib/outp/OverrideAndLimit  SystemSampleTime=-1  VariantActivationTime=update diagram  Latency=0  AutoFrameSizeCalculation=off
      link override Signal_Limit/_maxval: Value=KOUTP_CAASSwTimeOut_flg_maxval
      link override Signal_Limit/_minval: Value=KOUTP_CAASSwTimeOut_flg_minval
      link override Signal_Override/_ovrdflg: Value=KOUTP_CAASSwTimeOut_flg_ovrdflg
      link override Signal_Override/_ovrdval: Value=KOUTP_CAASSwTimeOut_flg_ovrdval
  VAPM_CAASSw_enum_Inproc : FVT_lib/outp/OverrideAndLimit  SystemSampleTime=-1  VariantActivationTime=update diagram  Latency=0  AutoFrameSizeCalculation=off
      link override Signal_Limit/_maxval: Value=KOUTP_CAASSw_enum_maxval
      link override Signal_Limit/_minval: Value=KOUTP_CAASSw_enum_minval
      link override Signal_Override/_ovrdflg: Value=KOUTP_CAASSw_enum_ovrdflg
      link override Signal_Override/_ovrdval: Value=KOUTP_CAASSw_enum_ovrdval
  VAPM_CAASVMCReqA_flg_Inproc : FVT_lib/outp/OverrideAndLimit  SystemSampleTime=-1  VariantActivationTime=update diagram  Latency=0  AutoFrameSizeCalculation=off
      link override Signal_Limit/_maxval: Value=KOUTP_CAASVMCReqA_flg_maxval
      link override Signal_Limit/_minval: Value=KOUTP_CAASVMCReqA_flg_minval
      link override Signal_Override/_ovrdflg: Value=KOUTP_CAASVMCReqA_flg_ovrdflg
      link override Signal_Override/_ovrdval: Value=KOUTP_CAASVMCReqA_flg_ovrdval
  VAPM_Chime_enum_Inproc : FVT_lib/outp/OverrideAndLimit  SystemSampleTime=-1  VariantActivationTime=update diagram  Latency=0  AutoFrameSizeCalculation=off
      link override Signal_Limit/_maxval: Value=KOUTP_Chime_enum_maxval
      link override Signal_Limit/_minval: Value=KOUTP_Chime_enum_minval
      link override Signal_Override/_ovrdflg: Value=KOUTP_Chime_enum_ovrdflg
      link override Signal_Override/_ovrdval: Value=KOUTP_Chime_enum_ovrdval
  VAPM_ChrgPlugSta_enum_Inproc : FVT_lib/outp/OverrideAndLimit  SystemSampleTime=-1  VariantActivationTime=update diagram  Latency=0  AutoFrameSizeCalculation=off
      link override Signal_Limit/_maxval: Value=KOUTP_ChrgPlugSta_enum_maxval
      link override Signal_Limit/_minval: Value=KOUTP_ChrgPlugSta_enum_minval
      link override Signal_Override/_ovrdflg: Value=KOUTP_ChrgPlugSta_enum_ovrdflg
      link override Signal_Override/_ovrdval: Value=KOUTP_ChrgPlugSta_enum_ovrdval
  VAPM_DKCPDkeyAreaRAPSSta_enum_Inproc : FVT_lib/outp/OverrideAndLimit  SystemSampleTime=-1  VariantActivationTime=update diagram  Latency=0  AutoFrameSizeCalculation=off
      link override Signal_Limit/_maxval: Value=KOUTP_DKCPDkeyAreaRAPSSta_enum_maxval
      link override Signal_Limit/_minval: Value=KOUTP_DKCPDkeyAreaRAPSSta_enum_minval
      link override Signal_Override/_ovrdflg: Value=KOUTP_DKCPDkeyAreaRAPSSta_enum_ovrdflg
      link override Signal_Override/_ovrdval: Value=KOUTP_DKCPDkeyAreaRAPSSta_enum_ovrdval
  VAPM_DKCParkingModeCmd_enum_Inproc : FVT_lib/outp/OverrideAndLimit  SystemSampleTime=-1  VariantActivationTime=update diagram  Latency=0  AutoFrameSizeCalculation=off
      link override Signal_Limit/_maxval: Value=KOUTP_DKCParkingModeCmd_enum_maxval
      link override Signal_Limit/_minval: Value=KOUTP_DKCParkingModeCmd_enum_minval
      link override Signal_Override/_ovrdflg: Value=KOUTP_DKCParkingModeCmd_enum_ovrdflg
      link override Signal_Override/_ovrdval: Value=KOUTP_DKCParkingModeCmd_enum_ovrdval
  VAPM_DriIntendTimeOut_flg_Inproc : FVT_lib/outp/OverrideAndLimit  SystemSampleTime=-1  VariantActivationTime=update diagram  Latency=0  AutoFrameSizeCalculation=off
      link override Signal_Limit/_maxval: Value=KOUTP_DriIntendTimeOut_flg_maxval
      link override Signal_Limit/_minval: Value=KOUTP_DriIntendTimeOut_flg_minval
      link override Signal_Override/_ovrdflg: Value=KOUTP_DriIntendTimeOut_flg_ovrdflg
      link override Signal_Override/_ovrdval: Value=KOUTP_DriIntendTimeOut_flg_ovrdval
  VAPM_DriIntend_enum_Inproc : FVT_lib/outp/OverrideAndLimit  SystemSampleTime=-1  VariantActivationTime=update diagram  Latency=0  AutoFrameSizeCalculation=off
      link override Signal_Limit/_maxval: Value=KOUTP_DriIntend_enum_maxval
      link override Signal_Limit/_minval: Value=KOUTP_DriIntend_enum_minval
      link override Signal_Override/_ovrdflg: Value=KOUTP_DriIntend_enum_ovrdflg
      link override Signal_Override/_ovrdval: Value=KOUTP_DriIntend_enum_ovrdval
  VAPM_DriverSeatBeltCmdTimeOut_flg_Inproc : FVT_lib/outp/OverrideAndLimit  SystemSampleTime=-1  VariantActivationTime=update diagram  Latency=0  AutoFrameSizeCalculation=off
      link override Signal_Limit/_maxval: Value=KOUTP_DriverSeatBeltCmdTimeOut_flg_maxval
      link override Signal_Limit/_minval: Value=KOUTP_DriverSeatBeltCmdTimeOut_flg_minval
      link override Signal_Override/_ovrdflg: Value=KOUTP_DriverSeatBeltCmdTimeOut_flg_ovrdflg
      link override Signal_Override/_ovrdval: Value=KOUTP_DriverSeatBeltCmdTimeOut_flg_ovrdval
  VAPM_DriverSeatBeltCmd_flg_Inproc : FVT_lib/outp/OverrideAndLimit  SystemSampleTime=-1  VariantActivationTime=update diagram  Latency=0  AutoFrameSizeCalculation=off
      link override Signal_Limit/_maxval: Value=KOUTP_DriverSeatBeltCmd_flg_maxval
      link override Signal_Limit/_minval: Value=KOUTP_DriverSeatBeltCmd_flg_minval
      link override Signal_Override/_ovrdflg: Value=KOUTP_DriverSeatBeltCmd_flg_ovrdflg
      link override Signal_Override/_ovrdval: Value=KOUTP_DriverSeatBeltCmd_flg_ovrdval
  VAPM_EPBErrStaTimeOut_flg_Inproc : FVT_lib/outp/OverrideAndLimit  SystemSampleTime=-1  VariantActivationTime=update diagram  Latency=0  AutoFrameSizeCalculation=off
      link override Signal_Limit/_maxval: Value=KOUTP_EPBErrStaTimeOut_flg_maxval
      link override Signal_Limit/_minval: Value=KOUTP_EPBErrStaTimeOut_flg_minval
      link override Signal_Override/_ovrdflg: Value=KOUTP_EPBErrStaTimeOut_flg_ovrdflg
      link override Signal_Override/_ovrdval: Value=KOUTP_EPBErrStaTimeOut_flg_ovrdval
  VAPM_EPBErrSta_enum_Inproc : FVT_lib/outp/OverrideAndLimit  SystemSampleTime=-1  VariantActivationTime=update diagram  Latency=0  AutoFrameSizeCalculation=off
      link override Signal_Limit/_maxval: Value=KOUTP_EPBErrSta_enum_maxval
      link override Signal_Limit/_minval: Value=KOUTP_EPBErrSta_enum_minval
      link override Signal_Override/_ovrdflg: Value=KOUTP_EPBErrSta_enum_ovrdflg
      link override Signal_Override/_ovrdval: Value=KOUTP_EPBErrSta_enum_ovrdval
  VAPM_EPBExtApplyAvailTimeOut_flg_Inproc : FVT_lib/outp/OverrideAndLimit  SystemSampleTime=-1  VariantActivationTime=update diagram  Latency=0  AutoFrameSizeCalculation=off
      link override Signal_Limit/_maxval: Value=KOUTP_EPBExtApplyAvailTimeOut_flg_maxval
      link override Signal_Limit/_minval: Value=KOUTP_EPBExtApplyAvailTimeOut_flg_minval
      link override Signal_Override/_ovrdflg: Value=KOUTP_EPBExtApplyAvailTimeOut_flg_ovrdflg
      link override Signal_Override/_ovrdval: Value=KOUTP_EPBExtApplyAvailTimeOut_flg_ovrdval
  VAPM_EPBExtApplyAvail_flg_Inproc : FVT_lib/outp/OverrideAndLimit  SystemSampleTime=-1  VariantActivationTime=update diagram  Latency=0  AutoFrameSizeCalculation=off
      link override Signal_Limit/_maxval: Value=KOUTP_EPBExtApplyAvail_flg_maxval
      link override Signal_Limit/_minval: Value=KOUTP_EPBExtApplyAvail_flg_minval
      link override Signal_Override/_ovrdflg: Value=KOUTP_EPBExtApplyAvail_flg_ovrdflg
      link override Signal_Override/_ovrdval: Value=KOUTP_EPBExtApplyAvail_flg_ovrdval
  VAPM_EPBExtReleaseAvailTimeOut_flg_Inproc : FVT_lib/outp/OverrideAndLimit  SystemSampleTime=-1  VariantActivationTime=update diagram  Latency=0  AutoFrameSizeCalculation=off
      link override Signal_Limit/_maxval: Value=KOUTP_EPBExtReleaseAvailTimeOut_flg_maxval
      link override Signal_Limit/_minval: Value=KOUTP_EPBExtReleaseAvailTimeOut_flg_minval
      link override Signal_Override/_ovrdflg: Value=KOUTP_EPBExtReleaseAvailTimeOut_flg_ovrdflg
      link override Signal_Override/_ovrdval: Value=KOUTP_EPBExtReleaseAvailTimeOut_flg_ovrdval
  VAPM_EPBExtReleaseAvail_flg_Inproc : FVT_lib/outp/OverrideAndLimit  SystemSampleTime=-1  VariantActivationTime=update diagram  Latency=0  AutoFrameSizeCalculation=off
      link override Signal_Limit/_maxval: Value=KOUTP_EPBExtReleaseAvail_flg_maxval
      link override Signal_Limit/_minval: Value=KOUTP_EPBExtReleaseAvail_flg_minval
      link override Signal_Override/_ovrdflg: Value=KOUTP_EPBExtReleaseAvail_flg_ovrdflg
      link override Signal_Override/_ovrdval: Value=KOUTP_EPBExtReleaseAvail_flg_ovrdval
  VAPM_EPBStaTimeOut_flg_Inproc : FVT_lib/outp/OverrideAndLimit  SystemSampleTime=-1  VariantActivationTime=update diagram  Latency=0  AutoFrameSizeCalculation=off
      link override Signal_Limit/_maxval: Value=KOUTP_EPBStaTimeOut_flg_maxval
      link override Signal_Limit/_minval: Value=KOUTP_EPBStaTimeOut_flg_minval
      link override Signal_Override/_ovrdflg: Value=KOUTP_EPBStaTimeOut_flg_ovrdflg
      link override Signal_Override/_ovrdval: Value=KOUTP_EPBStaTimeOut_flg_ovrdval
  VAPM_EPBSta_enum_Inproc : FVT_lib/outp/OverrideAndLimit  SystemSampleTime=-1  VariantActivationTime=update diagram  Latency=0  AutoFrameSizeCalculation=off
      link override Signal_Limit/_maxval: Value=KOUTP_EPBSta_enum_maxval
      link override Signal_Limit/_minval: Value=KOUTP_EPBSta_enum_minval
      link override Signal_Override/_ovrdflg: Value=KOUTP_EPBSta_enum_ovrdflg
      link override Signal_Override/_ovrdval: Value=KOUTP_EPBSta_enum_ovrdval
  VAPM_EPSAOIControlTimeOut_flg_Inproc : FVT_lib/outp/OverrideAndLimit  SystemSampleTime=-1  VariantActivationTime=update diagram  Latency=0  AutoFrameSizeCalculation=off
      link override Signal_Limit/_maxval: Value=KOUTP_EPSAOIControlTimeOut_flg_maxval
      link override Signal_Limit/_minval: Value=KOUTP_EPSAOIControlTimeOut_flg_minval
      link override Signal_Override/_ovrdflg: Value=KOUTP_EPSAOIControlTimeOut_flg_ovrdflg
      link override Signal_Override/_ovrdval: Value=KOUTP_EPSAOIControlTimeOut_flg_ovrdval
  VAPM_EPSAOIControl_enum_Inproc : FVT_lib/outp/OverrideAndLimit  SystemSampleTime=-1  VariantActivationTime=update diagram  Latency=0  AutoFrameSizeCalculation=off
      link override Signal_Limit/_maxval: Value=KOUTP_EPSAOIControl_enum_maxval
      link override Signal_Limit/_minval: Value=KOUTP_EPSAOIControl_enum_minval
      link override Signal_Override/_ovrdflg: Value=KOUTP_EPSAOIControl_enum_ovrdflg
      link override Signal_Override/_ovrdval: Value=KOUTP_EPSAOIControl_enum_ovrdval
  VAPM_ESCAPSStaTimeOut_flg_Inproc : FVT_lib/outp/OverrideAndLimit  SystemSampleTime=-1  VariantActivationTime=update diagram  Latency=0  AutoFrameSizeCalculation=off
      link override Signal_Limit/_maxval: Value=KOUTP_ESCAPSStaTimeOut_flg_maxval
      link override Signal_Limit/_minval: Value=KOUTP_ESCAPSStaTimeOut_flg_minval
      link override Signal_Override/_ovrdflg: Value=KOUTP_ESCAPSStaTimeOut_flg_ovrdflg
      link override Signal_Override/_ovrdval: Value=KOUTP_ESCAPSStaTimeOut_flg_ovrdval
  VAPM_ESCAPSSta_enum_Inproc : FVT_lib/outp/OverrideAndLimit  SystemSampleTime=-1  VariantActivationTime=update diagram  Latency=0  AutoFrameSizeCalculation=off
      link override Signal_Limit/_maxval: Value=KOUTP_ESCAPSSta_enum_maxval
      link override Signal_Limit/_minval: Value=KOUTP_ESCAPSSta_enum_minval
      link override Signal_Override/_ovrdflg: Value=KOUTP_ESCAPSSta_enum_ovrdflg
      link override Signal_Override/_ovrdval: Value=KOUTP_ESCAPSSta_enum_ovrdval
  VAPM_ESCStandstillTimeOut_flg_Inproc : FVT_lib/outp/OverrideAndLimit  SystemSampleTime=-1  VariantActivationTime=update diagram  Latency=0  AutoFrameSizeCalculation=off
      link override Signal_Limit/_maxval: Value=KOUTP_ESCStandstillTimeOut_flg_maxval
      link override Signal_Limit/_minval: Value=KOUTP_ESCStandstillTimeOut_flg_minval
      link override Signal_Override/_ovrdflg: Value=KOUTP_ESCStandstillTimeOut_flg_ovrdflg
      link override Signal_Override/_ovrdval: Value=KOUTP_ESCStandstillTimeOut_flg_ovrdval
  VAPM_ESCStandstill_flg_Inproc : FVT_lib/outp/OverrideAndLimit  SystemSampleTime=-1  VariantActivationTime=update diagram  Latency=0  AutoFrameSizeCalculation=off
      link override Signal_Limit/_maxval: Value=KOUTP_ESCStandstill_flg_maxval
      link override Signal_Limit/_minval: Value=KOUTP_ESCStandstill_flg_minval
      link override Signal_Override/_ovrdflg: Value=KOUTP_ESCStandstill_flg_ovrdflg
      link override Signal_Override/_ovrdval: Value=KOUTP_ESCStandstill_flg_ovrdval
  VAPM_FSOffSwTimeOut_flg_Inproc : FVT_lib/outp/OverrideAndLimit  SystemSampleTime=-1  VariantActivationTime=update diagram  Latency=0  AutoFrameSizeCalculation=off
      link override Signal_Limit/_maxval: Value=KOUTP_FSOffSwTimeOut_flg_maxval
      link override Signal_Limit/_minval: Value=KOUTP_FSOffSwTimeOut_flg_minval
      link override Signal_Override/_ovrdflg: Value=KOUTP_FSOffSwTimeOut_flg_ovrdflg
      link override Signal_Override/_ovrdval: Value=KOUTP_FSOffSwTimeOut_flg_ovrdval
  VAPM_FSOffSw_enum_Inproc : FVT_lib/outp/OverrideAndLimit  SystemSampleTime=-1  VariantActivationTime=update diagram  Latency=0  AutoFrameSizeCalculation=off
      link override Signal_Limit/_maxval: Value=KOUTP_FSOffSw_enum_maxval
      link override Signal_Limit/_minval: Value=KOUTP_FSOffSw_enum_minval
      link override Signal_Override/_ovrdflg: Value=KOUTP_FSOffSw_enum_ovrdflg
      link override Signal_Override/_ovrdval: Value=KOUTP_FSOffSw_enum_ovrdval
  VAPM_GRADETimeOut_flg_Inproc : FVT_lib/outp/OverrideAndLimit  SystemSampleTime=-1  VariantActivationTime=update diagram  Latency=0  AutoFrameSizeCalculation=off
      link override Signal_Limit/_maxval: Value=KOUTP_GRADETimeOut_flg_maxval
      link override Signal_Limit/_minval: Value=KOUTP_GRADETimeOut_flg_minval
      link override Signal_Override/_ovrdflg: Value=KOUTP_GRADETimeOut_flg_ovrdflg
      link override Signal_Override/_ovrdval: Value=KOUTP_GRADETimeOut_flg_ovrdval
  VAPM_GRADE_Deg_Inproc : FVT_lib/outp/OverrideAndLimit  SystemSampleTime=-1  VariantActivationTime=update diagram  Latency=0  AutoFrameSizeCalculation=off
      link override Signal_Limit/_maxval: Value=KOUTP_GRADE_Deg_maxval
      link override Signal_Limit/_minval: Value=KOUTP_GRADE_Deg_minval
      link override Signal_Override/_ovrdflg: Value=KOUTP_GRADE_Deg_ovrdflg
      link override Signal_Override/_ovrdval: Value=KOUTP_GRADE_Deg_ovrdval
  VAPM_IVIScreenTimeOut_flg_Inproc : FVT_lib/outp/OverrideAndLimit  SystemSampleTime=-1  VariantActivationTime=update diagram  Latency=0  AutoFrameSizeCalculation=off
      link override Signal_Limit/_maxval: Value=KOUTP_IVIScreenTimeOut_flg_maxval
      link override Signal_Limit/_minval: Value=KOUTP_IVIScreenTimeOut_flg_minval
      link override Signal_Override/_ovrdflg: Value=KOUTP_IVIScreenTimeOut_flg_ovrdflg
      link override Signal_Override/_ovrdval: Value=KOUTP_IVIScreenTimeOut_flg_ovrdval
  VAPM_IVIScreen_enum_Inproc : FVT_lib/outp/OverrideAndLimit  SystemSampleTime=-1  VariantActivationTime=update diagram  Latency=0  AutoFrameSizeCalculation=off
      link override Signal_Limit/_maxval: Value=KOUTP_IVIScreen_enum_maxval
      link override Signal_Limit/_minval: Value=KOUTP_IVIScreen_enum_minval
      link override Signal_Override/_ovrdflg: Value=KOUTP_IVIScreen_enum_ovrdflg
      link override Signal_Override/_ovrdval: Value=KOUTP_IVIScreen_enum_ovrdval
  VAPM_IVIStatusTimeOut_flg_Inproc : FVT_lib/outp/OverrideAndLimit  SystemSampleTime=-1  VariantActivationTime=update diagram  Latency=0  AutoFrameSizeCalculation=off
      link override Signal_Limit/_maxval: Value=KOUTP_IVIStatusTimeOut_flg_maxval
      link override Signal_Limit/_minval: Value=KOUTP_IVIStatusTimeOut_flg_minval
      link override Signal_Override/_ovrdflg: Value=KOUTP_IVIStatusTimeOut_flg_ovrdflg
      link override Signal_Override/_ovrdval: Value=KOUTP_IVIStatusTimeOut_flg_ovrdval
  VAPM_IVIStatus_flg_Inproc : FVT_lib/outp/OverrideAndLimit  SystemSampleTime=-1  VariantActivationTime=update diagram  Latency=0  AutoFrameSizeCalculation=off
      link override Signal_Limit/_maxval: Value=KOUTP_IVIStatus_flg_maxval
      link override Signal_Limit/_minval: Value=KOUTP_IVIStatus_flg_minval
      link override Signal_Override/_ovrdflg: Value=KOUTP_IVIStatus_flg_ovrdflg
      link override Signal_Override/_ovrdval: Value=KOUTP_IVIStatus_flg_ovrdval
  VAPM_IVIUserTakeOverAPSSta_flg_Inproc : FVT_lib/outp/OverrideAndLimit  SystemSampleTime=-1  VariantActivationTime=update diagram  Latency=0  AutoFrameSizeCalculation=off
      link override Signal_Limit/_maxval: Value=KOUTP_IVIUserTakeOverAPSSta_flg_maxval
      link override Signal_Limit/_minval: Value=KOUTP_IVIUserTakeOverAPSSta_flg_minval
      link override Signal_Override/_ovrdflg: Value=KOUTP_IVIUserTakeOverAPSSta_flg_ovrdflg
      link override Signal_Override/_ovrdval: Value=KOUTP_IVIUserTakeOverAPSSta_flg_ovrdval
  VAPM_LFPulseCountTimeOut_flg_Inproc : FVT_lib/outp/OverrideAndLimit  SystemSampleTime=-1  VariantActivationTime=update diagram  Latency=0  AutoFrameSizeCalculation=off
      link override Signal_Limit/_maxval: Value=KOUTP_LFPulseCountTimeOut_flg_maxval
      link override Signal_Limit/_minval: Value=KOUTP_LFPulseCountTimeOut_flg_minval
      link override Signal_Override/_ovrdflg: Value=KOUTP_LFPulseCountTimeOut_flg_ovrdflg
      link override Signal_Override/_ovrdval: Value=KOUTP_LFPulseCountTimeOut_flg_ovrdval
  VAPM_LFPulseCountVTimeOut_flg_Inproc : FVT_lib/outp/OverrideAndLimit  SystemSampleTime=-1  VariantActivationTime=update diagram  Latency=0  AutoFrameSizeCalculation=off
      link override Signal_Limit/_maxval: Value=KOUTP_LFPulseCountVTimeOut_flg_maxval
      link override Signal_Limit/_minval: Value=KOUTP_LFPulseCountVTimeOut_flg_minval
      link override Signal_Override/_ovrdflg: Value=KOUTP_LFPulseCountVTimeOut_flg_ovrdflg
      link override Signal_Override/_ovrdval: Value=KOUTP_LFPulseCountVTimeOut_flg_ovrdval
  VAPM_LFPulseCountV_flg_Inproc : FVT_lib/outp/OverrideAndLimit  SystemSampleTime=-1  VariantActivationTime=update diagram  Latency=0  AutoFrameSizeCalculation=off
      link override Signal_Limit/_maxval: Value=KOUTP_LFPulseCountV_flg_maxval
      link override Signal_Limit/_minval: Value=KOUTP_LFPulseCountV_flg_minval
      link override Signal_Override/_ovrdflg: Value=KOUTP_LFPulseCountV_flg_ovrdflg
      link override Signal_Override/_ovrdval: Value=KOUTP_LFPulseCountV_flg_ovrdval
  VAPM_LFPulseCount_enum_Inproc : FVT_lib/outp/OverrideAndLimit  SystemSampleTime=-1  VariantActivationTime=update diagram  Latency=0  AutoFrameSizeCalculation=off
      link override Signal_Limit/_maxval: Value=KOUTP_LFPulseCount_enum_maxval
      link override Signal_Limit/_minval: Value=KOUTP_LFPulseCount_enum_minval
      link override Signal_Override/_ovrdflg: Value=KOUTP_LFPulseCount_enum_ovrdflg
      link override Signal_Override/_ovrdval: Value=KOUTP_LFPulseCount_enum_ovrdval
  VAPM_LFRawWhlSpeedTimeOut_flg_Inproc : FVT_lib/outp/OverrideAndLimit  SystemSampleTime=-1  VariantActivationTime=update diagram  Latency=0  AutoFrameSizeCalculation=off
      link override Signal_Limit/_maxval: Value=KOUTP_LFRawWhlSpeedTimeOut_flg_maxval
      link override Signal_Limit/_minval: Value=KOUTP_LFRawWhlSpeedTimeOut_flg_minval
      link override Signal_Override/_ovrdflg: Value=KOUTP_LFRawWhlSpeedTimeOut_flg_ovrdflg
      link override Signal_Override/_ovrdval: Value=KOUTP_LFRawWhlSpeedTimeOut_flg_ovrdval
  VAPM_LFRawWhlSpeedVTimeOut_flg_Inproc : FVT_lib/outp/OverrideAndLimit  SystemSampleTime=-1  VariantActivationTime=update diagram  Latency=0  AutoFrameSizeCalculation=off
      link override Signal_Limit/_maxval: Value=KOUTP_LFRawWhlSpeedVTimeOut_flg_maxval
      link override Signal_Limit/_minval: Value=KOUTP_LFRawWhlSpeedVTimeOut_flg_minval
      link override Signal_Override/_ovrdflg: Value=KOUTP_LFRawWhlSpeedVTimeOut_flg_ovrdflg
      link override Signal_Override/_ovrdval: Value=KOUTP_LFRawWhlSpeedVTimeOut_flg_ovrdval
  VAPM_LFRawWhlSpeedV_flg_Inproc : FVT_lib/outp/OverrideAndLimit  SystemSampleTime=-1  VariantActivationTime=update diagram  Latency=0  AutoFrameSizeCalculation=off
      link override Signal_Limit/_maxval: Value=KOUTP_LFRawWhlSpeedV_flg_maxval
      link override Signal_Limit/_minval: Value=KOUTP_LFRawWhlSpeedV_flg_minval
      link override Signal_Override/_ovrdflg: Value=KOUTP_LFRawWhlSpeedV_flg_ovrdflg
      link override Signal_Override/_ovrdval: Value=KOUTP_LFRawWhlSpeedV_flg_ovrdval
  VAPM_LFRawWhlSpeed_kph_Inproc : FVT_lib/outp/OverrideAndLimit  SystemSampleTime=-1  VariantActivationTime=update diagram  Latency=0  AutoFrameSizeCalculation=off
      link override Signal_Limit/_maxval: Value=KOUTP_LFRawWhlSpeed_kph_maxval
      link override Signal_Limit/_minval: Value=KOUTP_LFRawWhlSpeed_kph_minval
      link override Signal_Override/_ovrdflg: Value=KOUTP_LFRawWhlSpeed_kph_ovrdflg
      link override Signal_Override/_ovrdval: Value=KOUTP_LFRawWhlSpeed_kph_ovrdval
  VAPM_LFWhlRotDirTimeOut_flg_Inproc : FVT_lib/outp/OverrideAndLimit  SystemSampleTime=-1  VariantActivationTime=update diagram  Latency=0  AutoFrameSizeCalculation=off
      link override Signal_Limit/_maxval: Value=KOUTP_LFWhlRotDirTimeOut_flg_maxval
      link override Signal_Limit/_minval: Value=KOUTP_LFWhlRotDirTimeOut_flg_minval
      link override Signal_Override/_ovrdflg: Value=KOUTP_LFWhlRotDirTimeOut_flg_ovrdflg
      link override Signal_Override/_ovrdval: Value=KOUTP_LFWhlRotDirTimeOut_flg_ovrdval
  VAPM_LFWhlRotDir_enum_Inproc : FVT_lib/outp/OverrideAndLimit  SystemSampleTime=-1  VariantActivationTime=update diagram  Latency=0  AutoFrameSizeCalculation=off
      link override Signal_Limit/_maxval: Value=KOUTP_LFWhlRotDir_enum_maxval
      link override Signal_Limit/_minval: Value=KOUTP_LFWhlRotDir_enum_minval
      link override Signal_Override/_ovrdflg: Value=KOUTP_LFWhlRotDir_enum_ovrdflg
      link override Signal_Override/_ovrdval: Value=KOUTP_LFWhlRotDir_enum_ovrdval
  VAPM_LRPulseCountTimeOut_flg_Inproc : FVT_lib/outp/OverrideAndLimit  SystemSampleTime=-1  VariantActivationTime=update diagram  Latency=0  AutoFrameSizeCalculation=off
      link override Signal_Limit/_maxval: Value=KOUTP_LRPulseCountTimeOut_flg_maxval
      link override Signal_Limit/_minval: Value=KOUTP_LRPulseCountTimeOut_flg_minval
      link override Signal_Override/_ovrdflg: Value=KOUTP_LRPulseCountTimeOut_flg_ovrdflg
      link override Signal_Override/_ovrdval: Value=KOUTP_LRPulseCountTimeOut_flg_ovrdval
  VAPM_LRPulseCountVTimeOut_flg_Inproc : FVT_lib/outp/OverrideAndLimit  SystemSampleTime=-1  VariantActivationTime=update diagram  Latency=0  AutoFrameSizeCalculation=off
      link override Signal_Limit/_maxval: Value=KOUTP_LRPulseCountVTimeOut_flg_maxval
      link override Signal_Limit/_minval: Value=KOUTP_LRPulseCountVTimeOut_flg_minval
      link override Signal_Override/_ovrdflg: Value=KOUTP_LRPulseCountVTimeOut_flg_ovrdflg
      link override Signal_Override/_ovrdval: Value=KOUTP_LRPulseCountVTimeOut_flg_ovrdval
  VAPM_LRPulseCountV_flg_Inproc : FVT_lib/outp/OverrideAndLimit  SystemSampleTime=-1  VariantActivationTime=update diagram  Latency=0  AutoFrameSizeCalculation=off
      link override Signal_Limit/_maxval: Value=KOUTP_LRPulseCountV_flg_maxval
      link override Signal_Limit/_minval: Value=KOUTP_LRPulseCountV_flg_minval
      link override Signal_Override/_ovrdflg: Value=KOUTP_LRPulseCountV_flg_ovrdflg
      link override Signal_Override/_ovrdval: Value=KOUTP_LRPulseCountV_flg_ovrdval
  VAPM_LRPulseCount_enum_Inproc : FVT_lib/outp/OverrideAndLimit  SystemSampleTime=-1  VariantActivationTime=update diagram  Latency=0  AutoFrameSizeCalculation=off
      link override Signal_Limit/_maxval: Value=KOUTP_LRPulseCount_enum_maxval
      link override Signal_Limit/_minval: Value=KOUTP_LRPulseCount_enum_minval
      link override Signal_Override/_ovrdflg: Value=KOUTP_LRPulseCount_enum_ovrdflg
      link override Signal_Override/_ovrdval: Value=KOUTP_LRPulseCount_enum_ovrdval
  VAPM_LRRawWhlSpeedTimeOut_flg_Inproc : FVT_lib/outp/OverrideAndLimit  SystemSampleTime=-1  VariantActivationTime=update diagram  Latency=0  AutoFrameSizeCalculation=off
      link override Signal_Limit/_maxval: Value=KOUTP_LRRawWhlSpeedTimeOut_flg_maxval
      link override Signal_Limit/_minval: Value=KOUTP_LRRawWhlSpeedTimeOut_flg_minval
      link override Signal_Override/_ovrdflg: Value=KOUTP_LRRawWhlSpeedTimeOut_flg_ovrdflg
      link override Signal_Override/_ovrdval: Value=KOUTP_LRRawWhlSpeedTimeOut_flg_ovrdval
  VAPM_LRRawWhlSpeedVTimeOut_flg_Inproc : FVT_lib/outp/OverrideAndLimit  SystemSampleTime=-1  VariantActivationTime=update diagram  Latency=0  AutoFrameSizeCalculation=off
      link override Signal_Limit/_maxval: Value=KOUTP_LRRawWhlSpeedVTimeOut_flg_maxval
      link override Signal_Limit/_minval: Value=KOUTP_LRRawWhlSpeedVTimeOut_flg_minval
      link override Signal_Override/_ovrdflg: Value=KOUTP_LRRawWhlSpeedVTimeOut_flg_ovrdflg
      link override Signal_Override/_ovrdval: Value=KOUTP_LRRawWhlSpeedVTimeOut_flg_ovrdval
  VAPM_LRRawWhlSpeedV_flg_Inproc : FVT_lib/outp/OverrideAndLimit  SystemSampleTime=-1  VariantActivationTime=update diagram  Latency=0  AutoFrameSizeCalculation=off
      link override Signal_Limit/_maxval: Value=KOUTP_LRRawWhlSpeedV_flg_maxval
      link override Signal_Limit/_minval: Value=KOUTP_LRRawWhlSpeedV_flg_minval
      link override Signal_Override/_ovrdflg: Value=KOUTP_LRRawWhlSpeedV_flg_ovrdflg
      link override Signal_Override/_ovrdval: Value=KOUTP_LRRawWhlSpeedV_flg_ovrdval
  VAPM_LRRawWhlSpeed_kph_Inproc : FVT_lib/outp/OverrideAndLimit  SystemSampleTime=-1  VariantActivationTime=update diagram  Latency=0  AutoFrameSizeCalculation=off
      link override Signal_Limit/_maxval: Value=KOUTP_LRRawWhlSpeed_kph_maxval
      link override Signal_Limit/_minval: Value=KOUTP_LRRawWhlSpeed_kph_minval
      link override Signal_Override/_ovrdflg: Value=KOUTP_LRRawWhlSpeed_kph_ovrdflg
      link override Signal_Override/_ovrdval: Value=KOUTP_LRRawWhlSpeed_kph_ovrdval
  VAPM_LRWhlRotDirTimeOut_flg_Inproc : FVT_lib/outp/OverrideAndLimit  SystemSampleTime=-1  VariantActivationTime=update diagram  Latency=0  AutoFrameSizeCalculation=off
      link override Signal_Limit/_maxval: Value=KOUTP_LRWhlRotDirTimeOut_flg_maxval
      link override Signal_Limit/_minval: Value=KOUTP_LRWhlRotDirTimeOut_flg_minval
      link override Signal_Override/_ovrdflg: Value=KOUTP_LRWhlRotDirTimeOut_flg_ovrdflg
      link override Signal_Override/_ovrdval: Value=KOUTP_LRWhlRotDirTimeOut_flg_ovrdval
  VAPM_LRWhlRotDir_enum_Inproc : FVT_lib/outp/OverrideAndLimit  SystemSampleTime=-1  VariantActivationTime=update diagram  Latency=0  AutoFrameSizeCalculation=off
      link override Signal_Limit/_maxval: Value=KOUTP_LRWhlRotDir_enum_maxval
      link override Signal_Limit/_minval: Value=KOUTP_LRWhlRotDir_enum_minval
      link override Signal_Override/_ovrdflg: Value=KOUTP_LRWhlRotDir_enum_ovrdflg
      link override Signal_Override/_ovrdval: Value=KOUTP_LRWhlRotDir_enum_ovrdval
  VAPM_LatAccelTimeOut_flg_Inproc : FVT_lib/outp/OverrideAndLimit  SystemSampleTime=-1  VariantActivationTime=update diagram  Latency=0  AutoFrameSizeCalculation=off
      link override Signal_Limit/_maxval: Value=KOUTP_LatAccelTimeOut_flg_maxval
      link override Signal_Limit/_minval: Value=KOUTP_LatAccelTimeOut_flg_minval
      link override Signal_Override/_ovrdflg: Value=KOUTP_LatAccelTimeOut_flg_ovrdflg
      link override Signal_Override/_ovrdval: Value=KOUTP_LatAccelTimeOut_flg_ovrdval
  VAPM_LatAccelVTimeOut_flg_Inproc : FVT_lib/outp/OverrideAndLimit  SystemSampleTime=-1  VariantActivationTime=update diagram  Latency=0  AutoFrameSizeCalculation=off
      link override Signal_Limit/_maxval: Value=KOUTP_LatAccelVTimeOut_flg_maxval
      link override Signal_Limit/_minval: Value=KOUTP_LatAccelVTimeOut_flg_minval
      link override Signal_Override/_ovrdflg: Value=KOUTP_LatAccelVTimeOut_flg_ovrdflg
      link override Signal_Override/_ovrdval: Value=KOUTP_LatAccelVTimeOut_flg_ovrdval
  VAPM_LatAccelV_flg_Inproc : FVT_lib/outp/OverrideAndLimit  SystemSampleTime=-1  VariantActivationTime=update diagram  Latency=0  AutoFrameSizeCalculation=off
      link override Signal_Limit/_maxval: Value=KOUTP_LatAccelV_flg_maxval
      link override Signal_Limit/_minval: Value=KOUTP_LatAccelV_flg_minval
      link override Signal_Override/_ovrdflg: Value=KOUTP_LatAccelV_flg_ovrdflg
      link override Signal_Override/_ovrdval: Value=KOUTP_LatAccelV_flg_ovrdval
  VAPM_LatAccel_Gps_Inproc : FVT_lib/outp/OverrideAndLimit  SystemSampleTime=-1  VariantActivationTime=update diagram  Latency=0  AutoFrameSizeCalculation=off
      link override Signal_Limit/_maxval: Value=KOUTP_LatAccel_Gps_maxval
      link override Signal_Limit/_minval: Value=KOUTP_LatAccel_Gps_minval
      link override Signal_Override/_ovrdflg: Value=KOUTP_LatAccel_Gps_ovrdflg
      link override Signal_Override/_ovrdval: Value=KOUTP_LatAccel_Gps_ovrdval
  VAPM_LongAccelTimeOut_flg_Inproc : FVT_lib/outp/OverrideAndLimit  SystemSampleTime=-1  VariantActivationTime=update diagram  Latency=0  AutoFrameSizeCalculation=off
      link override Signal_Limit/_maxval: Value=KOUTP_LongAccelTimeOut_flg_maxval
      link override Signal_Limit/_minval: Value=KOUTP_LongAccelTimeOut_flg_minval
      link override Signal_Override/_ovrdflg: Value=KOUTP_LongAccelTimeOut_flg_ovrdflg
      link override Signal_Override/_ovrdval: Value=KOUTP_LongAccelTimeOut_flg_ovrdval
  VAPM_LongAccelVTimeOut_flg_Inproc : FVT_lib/outp/OverrideAndLimit  SystemSampleTime=-1  VariantActivationTime=update diagram  Latency=0  AutoFrameSizeCalculation=off
      link override Signal_Limit/_maxval: Value=KOUTP_LongAccelVTimeOut_flg_maxval
      link override Signal_Limit/_minval: Value=KOUTP_LongAccelVTimeOut_flg_minval
      link override Signal_Override/_ovrdflg: Value=KOUTP_LongAccelVTimeOut_flg_ovrdflg
      link override Signal_Override/_ovrdval: Value=KOUTP_LongAccelVTimeOut_flg_ovrdval
  VAPM_LongAccelV_flg_Inproc : FVT_lib/outp/OverrideAndLimit  SystemSampleTime=-1  VariantActivationTime=update diagram  Latency=0  AutoFrameSizeCalculation=off
      link override Signal_Limit/_maxval: Value=KOUTP_LongAccelV_flg_maxval
      link override Signal_Limit/_minval: Value=KOUTP_LongAccelV_flg_minval
      link override Signal_Override/_ovrdflg: Value=KOUTP_LongAccelV_flg_ovrdflg
      link override Signal_Override/_ovrdval: Value=KOUTP_LongAccelV_flg_ovrdval
  VAPM_LongAccel_Gps_Inproc : FVT_lib/outp/OverrideAndLimit  SystemSampleTime=-1  VariantActivationTime=update diagram  Latency=0  AutoFrameSizeCalculation=off
      link override Signal_Limit/_maxval: Value=KOUTP_LongAccel_Gps_maxval
      link override Signal_Limit/_minval: Value=KOUTP_LongAccel_Gps_minval
      link override Signal_Override/_ovrdflg: Value=KOUTP_LongAccel_Gps_ovrdflg
      link override Signal_Override/_ovrdval: Value=KOUTP_LongAccel_Gps_ovrdval
  VAPM_MCPressureTimeOut_flg_Inproc : FVT_lib/outp/OverrideAndLimit  SystemSampleTime=-1  VariantActivationTime=update diagram  Latency=0  AutoFrameSizeCalculation=off
      link override Signal_Limit/_maxval: Value=KOUTP_MCPressureTimeOut_flg_maxval
      link override Signal_Limit/_minval: Value=KOUTP_MCPressureTimeOut_flg_minval
      link override Signal_Override/_ovrdflg: Value=KOUTP_MCPressureTimeOut_flg_ovrdflg
      link override Signal_Override/_ovrdval: Value=KOUTP_MCPressureTimeOut_flg_ovrdval
  VAPM_MCPressureVTimeOut_flg_Inproc : FVT_lib/outp/OverrideAndLimit  SystemSampleTime=-1  VariantActivationTime=update diagram  Latency=0  AutoFrameSizeCalculation=off
      link override Signal_Limit/_maxval: Value=KOUTP_MCPressureVTimeOut_flg_maxval
      link override Signal_Limit/_minval: Value=KOUTP_MCPressureVTimeOut_flg_minval
      link override Signal_Override/_ovrdflg: Value=KOUTP_MCPressureVTimeOut_flg_ovrdflg
      link override Signal_Override/_ovrdval: Value=KOUTP_MCPressureVTimeOut_flg_ovrdval
  VAPM_MCPressureV_bar_Inproc : FVT_lib/outp/OverrideAndLimit  SystemSampleTime=-1  VariantActivationTime=update diagram  Latency=0  AutoFrameSizeCalculation=off
      link override Signal_Limit/_maxval: Value=KOUTP_MCPressureV_bar_maxval
      link override Signal_Limit/_minval: Value=KOUTP_MCPressureV_bar_minval
      link override Signal_Override/_ovrdflg: Value=KOUTP_MCPressureV_bar_ovrdflg
      link override Signal_Override/_ovrdval: Value=KOUTP_MCPressureV_bar_ovrdval
  VAPM_MCPressure_bar_Inproc : FVT_lib/outp/OverrideAndLimit  SystemSampleTime=-1  VariantActivationTime=update diagram  Latency=0  AutoFrameSizeCalculation=off
      link override Signal_Limit/_maxval: Value=KOUTP_MCPressure_bar_maxval
      link override Signal_Limit/_minval: Value=KOUTP_MCPressure_bar_minval
      link override Signal_Override/_ovrdflg: Value=KOUTP_MCPressure_bar_ovrdflg
      link override Signal_Override/_ovrdval: Value=KOUTP_MCPressure_bar_ovrdval
  VAPM_ModOperation_enum_Inproc : FVT_lib/outp/OverrideAndLimit  SystemSampleTime=-1  VariantActivationTime=update diagram  Latency=0  AutoFrameSizeCalculation=off
      link override Signal_Limit/_maxval: Value=KOUTP_ModOperation_enum_maxval
      link override Signal_Limit/_minval: Value=KOUTP_ModOperation_enum_minval
      link override Signal_Override/_ovrdflg: Value=KOUTP_ModOperation_enum_ovrdflg
      link override Signal_Override/_ovrdval: Value=KOUTP_ModOperation_enum_ovrdval
  VAPM_PASAFCL_enum_Inproc : FVT_lib/outp/OverrideAndLimit  SystemSampleTime=-1  VariantActivationTime=update diagram  Latency=0  AutoFrameSizeCalculation=off
      link override Signal_Limit/_maxval: Value=KOUTP_PASAFCL_enum_maxval
      link override Signal_Limit/_minval: Value=KOUTP_PASAFCL_enum_minval
      link override Signal_Override/_ovrdflg: Value=KOUTP_PASAFCL_enum_ovrdflg
      link override Signal_Override/_ovrdval: Value=KOUTP_PASAFCL_enum_ovrdval
  VAPM_PASAFCR_enum_Inproc : FVT_lib/outp/OverrideAndLimit  SystemSampleTime=-1  VariantActivationTime=update diagram  Latency=0  AutoFrameSizeCalculation=off
      link override Signal_Limit/_maxval: Value=KOUTP_PASAFCR_enum_maxval
      link override Signal_Limit/_minval: Value=KOUTP_PASAFCR_enum_minval
      link override Signal_Override/_ovrdflg: Value=KOUTP_PASAFCR_enum_ovrdflg
      link override Signal_Override/_ovrdval: Value=KOUTP_PASAFCR_enum_ovrdval
  VAPM_PASAFML_enum_Inproc : FVT_lib/outp/OverrideAndLimit  SystemSampleTime=-1  VariantActivationTime=update diagram  Latency=0  AutoFrameSizeCalculation=off
      link override Signal_Limit/_maxval: Value=KOUTP_PASAFML_enum_maxval
      link override Signal_Limit/_minval: Value=KOUTP_PASAFML_enum_minval
      link override Signal_Override/_ovrdflg: Value=KOUTP_PASAFML_enum_ovrdflg
      link override Signal_Override/_ovrdval: Value=KOUTP_PASAFML_enum_ovrdval
  VAPM_PASAFMR_enum_Inproc : FVT_lib/outp/OverrideAndLimit  SystemSampleTime=-1  VariantActivationTime=update diagram  Latency=0  AutoFrameSizeCalculation=off
      link override Signal_Limit/_maxval: Value=KOUTP_PASAFMR_enum_maxval
      link override Signal_Limit/_minval: Value=KOUTP_PASAFMR_enum_minval
      link override Signal_Override/_ovrdflg: Value=KOUTP_PASAFMR_enum_ovrdflg
      link override Signal_Override/_ovrdval: Value=KOUTP_PASAFMR_enum_ovrdval
  VAPM_PASARCL_enum_Inproc : FVT_lib/outp/OverrideAndLimit  SystemSampleTime=-1  VariantActivationTime=update diagram  Latency=0  AutoFrameSizeCalculation=off
      link override Signal_Limit/_maxval: Value=KOUTP_PASARCL_enum_maxval
      link override Signal_Limit/_minval: Value=KOUTP_PASARCL_enum_minval
      link override Signal_Override/_ovrdflg: Value=KOUTP_PASARCL_enum_ovrdflg
      link override Signal_Override/_ovrdval: Value=KOUTP_PASARCL_enum_ovrdval
  VAPM_PASARCR_enum_Inproc : FVT_lib/outp/OverrideAndLimit  SystemSampleTime=-1  VariantActivationTime=update diagram  Latency=0  AutoFrameSizeCalculation=off
      link override Signal_Limit/_maxval: Value=KOUTP_PASARCR_enum_maxval
      link override Signal_Limit/_minval: Value=KOUTP_PASARCR_enum_minval
      link override Signal_Override/_ovrdflg: Value=KOUTP_PASARCR_enum_ovrdflg
      link override Signal_Override/_ovrdval: Value=KOUTP_PASARCR_enum_ovrdval
  VAPM_PASARML_enum_Inproc : FVT_lib/outp/OverrideAndLimit  SystemSampleTime=-1  VariantActivationTime=update diagram  Latency=0  AutoFrameSizeCalculation=off
      link override Signal_Limit/_maxval: Value=KOUTP_PASARML_enum_maxval
      link override Signal_Limit/_minval: Value=KOUTP_PASARML_enum_minval
      link override Signal_Override/_ovrdflg: Value=KOUTP_PASARML_enum_ovrdflg
      link override Signal_Override/_ovrdval: Value=KOUTP_PASARML_enum_ovrdval
  VAPM_PASARMR_enum_Inproc : FVT_lib/outp/OverrideAndLimit  SystemSampleTime=-1  VariantActivationTime=update diagram  Latency=0  AutoFrameSizeCalculation=off
      link override Signal_Limit/_maxval: Value=KOUTP_PASARMR_enum_maxval
      link override Signal_Limit/_minval: Value=KOUTP_PASARMR_enum_minval
      link override Signal_Override/_ovrdflg: Value=KOUTP_PASARMR_enum_ovrdflg
      link override Signal_Override/_ovrdval: Value=KOUTP_PASARMR_enum_ovrdval
  VAPM_PASDFCL_cm_Inproc : FVT_lib/outp/OverrideAndLimit  SystemSampleTime=-1  VariantActivationTime=update diagram  Latency=0  AutoFrameSizeCalculation=off
      link override Signal_Limit/_maxval: Value=KOUTP_PASDFCL_cm_maxval
      link override Signal_Limit/_minval: Value=KOUTP_PASDFCL_cm_minval
      link override Signal_Override/_ovrdflg: Value=KOUTP_PASDFCL_cm_ovrdflg
      link override Signal_Override/_ovrdval: Value=KOUTP_PASDFCL_cm_ovrdval
  VAPM_PASDFCR_cm_Inproc : FVT_lib/outp/OverrideAndLimit  SystemSampleTime=-1  VariantActivationTime=update diagram  Latency=0  AutoFrameSizeCalculation=off
      link override Signal_Limit/_maxval: Value=KOUTP_PASDFCR_cm_maxval
      link override Signal_Limit/_minval: Value=KOUTP_PASDFCR_cm_minval
      link override Signal_Override/_ovrdflg: Value=KOUTP_PASDFCR_cm_ovrdflg
      link override Signal_Override/_ovrdval: Value=KOUTP_PASDFCR_cm_ovrdval
  VAPM_PASDFML_cm_Inproc : FVT_lib/outp/OverrideAndLimit  SystemSampleTime=-1  VariantActivationTime=update diagram  Latency=0  AutoFrameSizeCalculation=off
      link override Signal_Limit/_maxval: Value=KOUTP_PASDFML_cm_maxval
      link override Signal_Limit/_minval: Value=KOUTP_PASDFML_cm_minval
      link override Signal_Override/_ovrdflg: Value=KOUTP_PASDFML_cm_ovrdflg
      link override Signal_Override/_ovrdval: Value=KOUTP_PASDFML_cm_ovrdval
  VAPM_PASDFMR_cm_Inproc : FVT_lib/outp/OverrideAndLimit  SystemSampleTime=-1  VariantActivationTime=update diagram  Latency=0  AutoFrameSizeCalculation=off
      link override Signal_Limit/_maxval: Value=KOUTP_PASDFMR_cm_maxval
      link override Signal_Limit/_minval: Value=KOUTP_PASDFMR_cm_minval
      link override Signal_Override/_ovrdflg: Value=KOUTP_PASDFMR_cm_ovrdflg
      link override Signal_Override/_ovrdval: Value=KOUTP_PASDFMR_cm_ovrdval
  VAPM_PASDRCL_cm_Inproc : FVT_lib/outp/OverrideAndLimit  SystemSampleTime=-1  VariantActivationTime=update diagram  Latency=0  AutoFrameSizeCalculation=off
      link override Signal_Limit/_maxval: Value=KOUTP_PASDRCL_cm_maxval
      link override Signal_Limit/_minval: Value=KOUTP_PASDRCL_cm_minval
      link override Signal_Override/_ovrdflg: Value=KOUTP_PASDRCL_cm_ovrdflg
      link override Signal_Override/_ovrdval: Value=KOUTP_PASDRCL_cm_ovrdval
  VAPM_PASDRCR_cm_Inproc : FVT_lib/outp/OverrideAndLimit  SystemSampleTime=-1  VariantActivationTime=update diagram  Latency=0  AutoFrameSizeCalculation=off
      link override Signal_Limit/_maxval: Value=KOUTP_PASDRCR_cm_maxval
      link override Signal_Limit/_minval: Value=KOUTP_PASDRCR_cm_minval
      link override Signal_Override/_ovrdflg: Value=KOUTP_PASDRCR_cm_ovrdflg
      link override Signal_Override/_ovrdval: Value=KOUTP_PASDRCR_cm_ovrdval
  VAPM_PASDRML_cm_Inproc : FVT_lib/outp/OverrideAndLimit  SystemSampleTime=-1  VariantActivationTime=update diagram  Latency=0  AutoFrameSizeCalculation=off
      link override Signal_Limit/_maxval: Value=KOUTP_PASDRML_cm_maxval
      link override Signal_Limit/_minval: Value=KOUTP_PASDRML_cm_minval
      link override Signal_Override/_ovrdflg: Value=KOUTP_PASDRML_cm_ovrdflg
      link override Signal_Override/_ovrdval: Value=KOUTP_PASDRML_cm_ovrdval
  VAPM_PASDRMR_cm_Inproc : FVT_lib/outp/OverrideAndLimit  SystemSampleTime=-1  VariantActivationTime=update diagram  Latency=0  AutoFrameSizeCalculation=off
      link override Signal_Limit/_maxval: Value=KOUTP_PASDRMR_cm_maxval
      link override Signal_Limit/_minval: Value=KOUTP_PASDRMR_cm_minval
      link override Signal_Override/_ovrdflg: Value=KOUTP_PASDRMR_cm_ovrdflg
      link override Signal_Override/_ovrdval: Value=KOUTP_PASDRMR_cm_ovrdval
  VAPM_PUIDLowPower_flg_Inproc : FVT_lib/outp/OverrideAndLimit  SystemSampleTime=-1  VariantActivationTime=update diagram  Latency=0  AutoFrameSizeCalculation=off
      link override Signal_Limit/_maxval: Value=KOUTP_PUIDLowPower_flg_maxval
      link override Signal_Limit/_minval: Value=KOUTP_PUIDLowPower_flg_minval
      link override Signal_Override/_ovrdflg: Value=KOUTP_PUIDLowPower_flg_ovrdflg
      link override Signal_Override/_ovrdval: Value=KOUTP_PUIDLowPower_flg_ovrdval
  VAPM_RAPSBCMLamp_enum_Inproc : FVT_lib/outp/OverrideAndLimit  SystemSampleTime=-1  VariantActivationTime=update diagram  Latency=0  AutoFrameSizeCalculation=off
      link override Signal_Limit/_maxval: Value=KOUTP_RAPSBCMLamp_enum_maxval
      link override Signal_Limit/_minval: Value=KOUTP_RAPSBCMLamp_enum_minval
      link override Signal_Override/_ovrdflg: Value=KOUTP_RAPSBCMLamp_enum_ovrdflg
      link override Signal_Override/_ovrdval: Value=KOUTP_RAPSBCMLamp_enum_ovrdval
  VAPM_RAPSBCMLockReq_flg_Inproc : FVT_lib/outp/OverrideAndLimit  SystemSampleTime=-1  VariantActivationTime=update diagram  Latency=0  AutoFrameSizeCalculation=off
      link override Signal_Limit/_maxval: Value=KOUTP_RAPSBCMLockReq_flg_maxval
      link override Signal_Limit/_minval: Value=KOUTP_RAPSBCMLockReq_flg_minval
      link override Signal_Override/_ovrdflg: Value=KOUTP_RAPSBCMLockReq_flg_ovrdflg
      link override Signal_Override/_ovrdval: Value=KOUTP_RAPSBCMLockReq_flg_ovrdval
  VAPM_RAPSErrLv1_flg_Inproc : FVT_lib/outp/OverrideAndLimit  SystemSampleTime=-1  VariantActivationTime=update diagram  Latency=0  AutoFrameSizeCalculation=off
      link override Signal_Limit/_maxval: Value=KOUTP_RAPSErrLv1_flg_maxval
      link override Signal_Limit/_minval: Value=KOUTP_RAPSErrLv1_flg_minval
      link override Signal_Override/_ovrdflg: Value=KOUTP_RAPSErrLv1_flg_ovrdflg
      link override Signal_Override/_ovrdval: Value=KOUTP_RAPSErrLv1_flg_ovrdval
  VAPM_RAPSErrWarnSta_enum_Inproc : FVT_lib/outp/OverrideAndLimit  SystemSampleTime=-1  VariantActivationTime=update diagram  Latency=0  AutoFrameSizeCalculation=off
      link override Signal_Limit/_maxval: Value=KOUTP_RAPSErrWarnSta_enum_maxval
      link override Signal_Limit/_minval: Value=KOUTP_RAPSErrWarnSta_enum_minval
      link override Signal_Override/_ovrdflg: Value=KOUTP_RAPSErrWarnSta_enum_ovrdflg
      link override Signal_Override/_ovrdval: Value=KOUTP_RAPSErrWarnSta_enum_ovrdval
  VAPM_RFPulseCountTimeOut_flg_Inproc : FVT_lib/outp/OverrideAndLimit  SystemSampleTime=-1  VariantActivationTime=update diagram  Latency=0  AutoFrameSizeCalculation=off
      link override Signal_Limit/_maxval: Value=KOUTP_RFPulseCountTimeOut_flg_maxval
      link override Signal_Limit/_minval: Value=KOUTP_RFPulseCountTimeOut_flg_minval
      link override Signal_Override/_ovrdflg: Value=KOUTP_RFPulseCountTimeOut_flg_ovrdflg
      link override Signal_Override/_ovrdval: Value=KOUTP_RFPulseCountTimeOut_flg_ovrdval
  VAPM_RFPulseCountVTimeOut_flg_Inproc : FVT_lib/outp/OverrideAndLimit  SystemSampleTime=-1  VariantActivationTime=update diagram  Latency=0  AutoFrameSizeCalculation=off
      link override Signal_Limit/_maxval: Value=KOUTP_RFPulseCountVTimeOut_flg_maxval
      link override Signal_Limit/_minval: Value=KOUTP_RFPulseCountVTimeOut_flg_minval
      link override Signal_Override/_ovrdflg: Value=KOUTP_RFPulseCountVTimeOut_flg_ovrdflg
      link override Signal_Override/_ovrdval: Value=KOUTP_RFPulseCountVTimeOut_flg_ovrdval
  VAPM_RFPulseCountV_flg_Inproc : FVT_lib/outp/OverrideAndLimit  SystemSampleTime=-1  VariantActivationTime=update diagram  Latency=0  AutoFrameSizeCalculation=off
      link override Signal_Limit/_maxval: Value=KOUTP_RFPulseCountV_flg_maxval
      link override Signal_Limit/_minval: Value=KOUTP_RFPulseCountV_flg_minval
      link override Signal_Override/_ovrdflg: Value=KOUTP_RFPulseCountV_flg_ovrdflg
      link override Signal_Override/_ovrdval: Value=KOUTP_RFPulseCountV_flg_ovrdval
  VAPM_RFPulseCount_enum_Inproc : FVT_lib/outp/OverrideAndLimit  SystemSampleTime=-1  VariantActivationTime=update diagram  Latency=0  AutoFrameSizeCalculation=off
      link override Signal_Limit/_maxval: Value=KOUTP_RFPulseCount_enum_maxval
      link override Signal_Limit/_minval: Value=KOUTP_RFPulseCount_enum_minval
      link override Signal_Override/_ovrdflg: Value=KOUTP_RFPulseCount_enum_ovrdflg
      link override Signal_Override/_ovrdval: Value=KOUTP_RFPulseCount_enum_ovrdval
  VAPM_RFRawWhlSpeedTimeOut_flg_Inproc : FVT_lib/outp/OverrideAndLimit  SystemSampleTime=-1  VariantActivationTime=update diagram  Latency=0  AutoFrameSizeCalculation=off
      link override Signal_Limit/_maxval: Value=KOUTP_RFRawWhlSpeedTimeOut_flg_maxval
      link override Signal_Limit/_minval: Value=KOUTP_RFRawWhlSpeedTimeOut_flg_minval
      link override Signal_Override/_ovrdflg: Value=KOUTP_RFRawWhlSpeedTimeOut_flg_ovrdflg
      link override Signal_Override/_ovrdval: Value=KOUTP_RFRawWhlSpeedTimeOut_flg_ovrdval
  VAPM_RFRawWhlSpeedVTimeOut_flg_Inproc : FVT_lib/outp/OverrideAndLimit  SystemSampleTime=-1  VariantActivationTime=update diagram  Latency=0  AutoFrameSizeCalculation=off
      link override Signal_Limit/_maxval: Value=KOUTP_RFRawWhlSpeedVTimeOut_flg_maxval
      link override Signal_Limit/_minval: Value=KOUTP_RFRawWhlSpeedVTimeOut_flg_minval
      link override Signal_Override/_ovrdflg: Value=KOUTP_RFRawWhlSpeedVTimeOut_flg_ovrdflg
      link override Signal_Override/_ovrdval: Value=KOUTP_RFRawWhlSpeedVTimeOut_flg_ovrdval
  VAPM_RFRawWhlSpeedV_flg_Inproc : FVT_lib/outp/OverrideAndLimit  SystemSampleTime=-1  VariantActivationTime=update diagram  Latency=0  AutoFrameSizeCalculation=off
      link override Signal_Limit/_maxval: Value=KOUTP_RFRawWhlSpeedV_flg_maxval
      link override Signal_Limit/_minval: Value=KOUTP_RFRawWhlSpeedV_flg_minval
      link override Signal_Override/_ovrdflg: Value=KOUTP_RFRawWhlSpeedV_flg_ovrdflg
      link override Signal_Override/_ovrdval: Value=KOUTP_RFRawWhlSpeedV_flg_ovrdval
  VAPM_RFRawWhlSpeed_kph_Inproc : FVT_lib/outp/OverrideAndLimit  SystemSampleTime=-1  VariantActivationTime=update diagram  Latency=0  AutoFrameSizeCalculation=off
      link override Signal_Limit/_maxval: Value=KOUTP_RFRawWhlSpeed_kph_maxval
      link override Signal_Limit/_minval: Value=KOUTP_RFRawWhlSpeed_kph_minval
      link override Signal_Override/_ovrdflg: Value=KOUTP_RFRawWhlSpeed_kph_ovrdflg
      link override Signal_Override/_ovrdval: Value=KOUTP_RFRawWhlSpeed_kph_ovrdval
  VAPM_RFWhlRotDirTimeOut_flg_Inproc : FVT_lib/outp/OverrideAndLimit  SystemSampleTime=-1  VariantActivationTime=update diagram  Latency=0  AutoFrameSizeCalculation=off
      link override Signal_Limit/_maxval: Value=KOUTP_RFWhlRotDirTimeOut_flg_maxval
      link override Signal_Limit/_minval: Value=KOUTP_RFWhlRotDirTimeOut_flg_minval
      link override Signal_Override/_ovrdflg: Value=KOUTP_RFWhlRotDirTimeOut_flg_ovrdflg
      link override Signal_Override/_ovrdval: Value=KOUTP_RFWhlRotDirTimeOut_flg_ovrdval
  VAPM_RFWhlRotDir_enum_Inproc : FVT_lib/outp/OverrideAndLimit  SystemSampleTime=-1  VariantActivationTime=update diagram  Latency=0  AutoFrameSizeCalculation=off
      link override Signal_Limit/_maxval: Value=KOUTP_RFWhlRotDir_enum_maxval
      link override Signal_Limit/_minval: Value=KOUTP_RFWhlRotDir_enum_minval
      link override Signal_Override/_ovrdflg: Value=KOUTP_RFWhlRotDir_enum_ovrdflg
      link override Signal_Override/_ovrdval: Value=KOUTP_RFWhlRotDir_enum_ovrdval
  VAPM_RRPulseCountTimeOut_flg_Inproc : FVT_lib/outp/OverrideAndLimit  SystemSampleTime=-1  VariantActivationTime=update diagram  Latency=0  AutoFrameSizeCalculation=off
      link override Signal_Limit/_maxval: Value=KOUTP_RRPulseCountTimeOut_flg_maxval
      link override Signal_Limit/_minval: Value=KOUTP_RRPulseCountTimeOut_flg_minval
      link override Signal_Override/_ovrdflg: Value=KOUTP_RRPulseCountTimeOut_flg_ovrdflg
      link override Signal_Override/_ovrdval: Value=KOUTP_RRPulseCountTimeOut_flg_ovrdval
  VAPM_RRPulseCountVTimeOut_flg_Inproc : FVT_lib/outp/OverrideAndLimit  SystemSampleTime=-1  VariantActivationTime=update diagram  Latency=0  AutoFrameSizeCalculation=off
      link override Signal_Limit/_maxval: Value=KOUTP_RRPulseCountVTimeOut_flg_maxval
      link override Signal_Limit/_minval: Value=KOUTP_RRPulseCountVTimeOut_flg_minval
      link override Signal_Override/_ovrdflg: Value=KOUTP_RRPulseCountVTimeOut_flg_ovrdflg
      link override Signal_Override/_ovrdval: Value=KOUTP_RRPulseCountVTimeOut_flg_ovrdval
  VAPM_RRPulseCountV_flg_Inproc : FVT_lib/outp/OverrideAndLimit  SystemSampleTime=-1  VariantActivationTime=update diagram  Latency=0  AutoFrameSizeCalculation=off
      link override Signal_Limit/_maxval: Value=KOUTP_RRPulseCountV_flg_maxval
      link override Signal_Limit/_minval: Value=KOUTP_RRPulseCountV_flg_minval
      link override Signal_Override/_ovrdflg: Value=KOUTP_RRPulseCountV_flg_ovrdflg
      link override Signal_Override/_ovrdval: Value=KOUTP_RRPulseCountV_flg_ovrdval
  VAPM_RRPulseCount_enum_Inproc : FVT_lib/outp/OverrideAndLimit  SystemSampleTime=-1  VariantActivationTime=update diagram  Latency=0  AutoFrameSizeCalculation=off
      link override Signal_Limit/_maxval: Value=KOUTP_RRPulseCount_enum_maxval
      link override Signal_Limit/_minval: Value=KOUTP_RRPulseCount_enum_minval
      link override Signal_Override/_ovrdflg: Value=KOUTP_RRPulseCount_enum_ovrdflg
      link override Signal_Override/_ovrdval: Value=KOUTP_RRPulseCount_enum_ovrdval
  VAPM_RRRawWhlSpeedTimeOut_flg_Inproc : FVT_lib/outp/OverrideAndLimit  SystemSampleTime=-1  VariantActivationTime=update diagram  Latency=0  AutoFrameSizeCalculation=off
      link override Signal_Limit/_maxval: Value=KOUTP_RRRawWhlSpeedTimeOut_flg_maxval
      link override Signal_Limit/_minval: Value=KOUTP_RRRawWhlSpeedTimeOut_flg_minval
      link override Signal_Override/_ovrdflg: Value=KOUTP_RRRawWhlSpeedTimeOut_flg_ovrdflg
      link override Signal_Override/_ovrdval: Value=KOUTP_RRRawWhlSpeedTimeOut_flg_ovrdval
  VAPM_RRRawWhlSpeedVTimeOut_flg_Inproc : FVT_lib/outp/OverrideAndLimit  SystemSampleTime=-1  VariantActivationTime=update diagram  Latency=0  AutoFrameSizeCalculation=off
      link override Signal_Limit/_maxval: Value=KOUTP_RRRawWhlSpeedVTimeOut_flg_maxval
      link override Signal_Limit/_minval: Value=KOUTP_RRRawWhlSpeedVTimeOut_flg_minval
      link override Signal_Override/_ovrdflg: Value=KOUTP_RRRawWhlSpeedVTimeOut_flg_ovrdflg
      link override Signal_Override/_ovrdval: Value=KOUTP_RRRawWhlSpeedVTimeOut_flg_ovrdval
  VAPM_RRRawWhlSpeedV_flg_Inproc : FVT_lib/outp/OverrideAndLimit  SystemSampleTime=-1  VariantActivationTime=update diagram  Latency=0  AutoFrameSizeCalculation=off
      link override Signal_Limit/_maxval: Value=KOUTP_RRRawWhlSpeedV_flg_maxval
      link override Signal_Limit/_minval: Value=KOUTP_RRRawWhlSpeedV_flg_minval
      link override Signal_Override/_ovrdflg: Value=KOUTP_RRRawWhlSpeedV_flg_ovrdflg
      link override Signal_Override/_ovrdval: Value=KOUTP_RRRawWhlSpeedV_flg_ovrdval
  VAPM_RRRawWhlSpeed_kph_Inproc : FVT_lib/outp/OverrideAndLimit  SystemSampleTime=-1  VariantActivationTime=update diagram  Latency=0  AutoFrameSizeCalculation=off
      link override Signal_Limit/_maxval: Value=KOUTP_RRRawWhlSpeed_kph_maxval
      link override Signal_Limit/_minval: Value=KOUTP_RRRawWhlSpeed_kph_minval
      link override Signal_Override/_ovrdflg: Value=KOUTP_RRRawWhlSpeed_kph_ovrdflg
      link override Signal_Override/_ovrdval: Value=KOUTP_RRRawWhlSpeed_kph_ovrdval
  VAPM_RRWhlRotDirTimeOut_flg_Inproc : FVT_lib/outp/OverrideAndLimit  SystemSampleTime=-1  VariantActivationTime=update diagram  Latency=0  AutoFrameSizeCalculation=off
      link override Signal_Limit/_maxval: Value=KOUTP_RRWhlRotDirTimeOut_flg_maxval
      link override Signal_Limit/_minval: Value=KOUTP_RRWhlRotDirTimeOut_flg_minval
      link override Signal_Override/_ovrdflg: Value=KOUTP_RRWhlRotDirTimeOut_flg_ovrdflg
      link override Signal_Override/_ovrdval: Value=KOUTP_RRWhlRotDirTimeOut_flg_ovrdval
  VAPM_RRWhlRotDir_enum_Inproc : FVT_lib/outp/OverrideAndLimit  SystemSampleTime=-1  VariantActivationTime=update diagram  Latency=0  AutoFrameSizeCalculation=off
      link override Signal_Limit/_maxval: Value=KOUTP_RRWhlRotDir_enum_maxval
      link override Signal_Limit/_minval: Value=KOUTP_RRWhlRotDir_enum_minval
      link override Signal_Override/_ovrdflg: Value=KOUTP_RRWhlRotDir_enum_ovrdflg
      link override Signal_Override/_ovrdval: Value=KOUTP_RRWhlRotDir_enum_ovrdval
  VAPM_SASAngleTimeOut_flg_Inproc : FVT_lib/outp/OverrideAndLimit  SystemSampleTime=-1  VariantActivationTime=update diagram  Latency=0  AutoFrameSizeCalculation=off
      link override Signal_Limit/_maxval: Value=KOUTP_SASAngleTimeOut_flg_maxval
      link override Signal_Limit/_minval: Value=KOUTP_SASAngleTimeOut_flg_minval
      link override Signal_Override/_ovrdflg: Value=KOUTP_SASAngleTimeOut_flg_ovrdflg
      link override Signal_Override/_ovrdval: Value=KOUTP_SASAngleTimeOut_flg_ovrdval
  VAPM_SASAngle_Deg_Inproc : FVT_lib/outp/OverrideAndLimit  SystemSampleTime=-1  VariantActivationTime=update diagram  Latency=0  AutoFrameSizeCalculation=off
      link override Signal_Limit/_maxval: Value=KOUTP_SASAngle_Deg_maxval
      link override Signal_Limit/_minval: Value=KOUTP_SASAngle_Deg_minval
      link override Signal_Override/_ovrdflg: Value=KOUTP_SASAngle_Deg_ovrdflg
      link override Signal_Override/_ovrdval: Value=KOUTP_SASAngle_Deg_ovrdval
  VAPM_SASCALTimeOut_flg_Inproc : FVT_lib/outp/OverrideAndLimit  SystemSampleTime=-1  VariantActivationTime=update diagram  Latency=0  AutoFrameSizeCalculation=off
      link override Signal_Limit/_maxval: Value=KOUTP_SASCALTimeOut_flg_maxval
      link override Signal_Limit/_minval: Value=KOUTP_SASCALTimeOut_flg_minval
      link override Signal_Override/_ovrdflg: Value=KOUTP_SASCALTimeOut_flg_ovrdflg
      link override Signal_Override/_ovrdval: Value=KOUTP_SASCALTimeOut_flg_ovrdval
  VAPM_SASCAL_flg_Inproc : FVT_lib/outp/OverrideAndLimit  SystemSampleTime=-1  VariantActivationTime=update diagram  Latency=0  AutoFrameSizeCalculation=off
      link override Signal_Limit/_maxval: Value=KOUTP_SASCAL_flg_maxval
      link override Signal_Limit/_minval: Value=KOUTP_SASCAL_flg_minval
      link override Signal_Override/_ovrdflg: Value=KOUTP_SASCAL_flg_ovrdflg
      link override Signal_Override/_ovrdval: Value=KOUTP_SASCAL_flg_ovrdval
  VAPM_SASSpeedTimeOut_flg_Inproc : FVT_lib/outp/OverrideAndLimit  SystemSampleTime=-1  VariantActivationTime=update diagram  Latency=0  AutoFrameSizeCalculation=off
      link override Signal_Limit/_maxval: Value=KOUTP_SASSpeedTimeOut_flg_maxval
      link override Signal_Limit/_minval: Value=KOUTP_SASSpeedTimeOut_flg_minval
      link override Signal_Override/_ovrdflg: Value=KOUTP_SASSpeedTimeOut_flg_ovrdflg
      link override Signal_Override/_ovrdval: Value=KOUTP_SASSpeedTimeOut_flg_ovrdval
  VAPM_SASSpeedValidTimeOut_flg_Inproc : FVT_lib/outp/OverrideAndLimit  SystemSampleTime=-1  VariantActivationTime=update diagram  Latency=0  AutoFrameSizeCalculation=off
      link override Signal_Limit/_maxval: Value=KOUTP_SASSpeedValidTimeOut_flg_maxval
      link override Signal_Limit/_minval: Value=KOUTP_SASSpeedValidTimeOut_flg_minval
      link override Signal_Override/_ovrdflg: Value=KOUTP_SASSpeedValidTimeOut_flg_ovrdflg
      link override Signal_Override/_ovrdval: Value=KOUTP_SASSpeedValidTimeOut_flg_ovrdval
  VAPM_SASSpeedValid_flg_Inproc : FVT_lib/outp/OverrideAndLimit  SystemSampleTime=-1  VariantActivationTime=update diagram  Latency=0  AutoFrameSizeCalculation=off
      link override Signal_Limit/_maxval: Value=KOUTP_SASSpeedValid_flg_maxval
      link override Signal_Limit/_minval: Value=KOUTP_SASSpeedValid_flg_minval
      link override Signal_Override/_ovrdflg: Value=KOUTP_SASSpeedValid_flg_ovrdflg
      link override Signal_Override/_ovrdval: Value=KOUTP_SASSpeedValid_flg_ovrdval
  VAPM_SASSpeed_degps_Inproc : FVT_lib/outp/OverrideAndLimit  SystemSampleTime=-1  VariantActivationTime=update diagram  Latency=0  AutoFrameSizeCalculation=off
      link override Signal_Limit/_maxval: Value=KOUTP_SASSpeed_degps_maxval
      link override Signal_Limit/_minval: Value=KOUTP_SASSpeed_degps_minval
      link override Signal_Override/_ovrdflg: Value=KOUTP_SASSpeed_degps_ovrdflg
      link override Signal_Override/_ovrdval: Value=KOUTP_SASSpeed_degps_ovrdval
  VAPM_SASVTimeOut_flg_Inproc : FVT_lib/outp/OverrideAndLimit  SystemSampleTime=-1  VariantActivationTime=update diagram  Latency=0  AutoFrameSizeCalculation=off
      link override Signal_Limit/_maxval: Value=KOUTP_SASVTimeOut_flg_maxval
      link override Signal_Limit/_minval: Value=KOUTP_SASVTimeOut_flg_minval
      link override Signal_Override/_ovrdflg: Value=KOUTP_SASVTimeOut_flg_ovrdflg
      link override Signal_Override/_ovrdval: Value=KOUTP_SASVTimeOut_flg_ovrdval
  VAPM_SASV_flg_Inproc : FVT_lib/outp/OverrideAndLimit  SystemSampleTime=-1  VariantActivationTime=update diagram  Latency=0  AutoFrameSizeCalculation=off
      link override Signal_Limit/_maxval: Value=KOUTP_SASV_flg_maxval
      link override Signal_Limit/_minval: Value=KOUTP_SASV_flg_minval
      link override Signal_Override/_ovrdflg: Value=KOUTP_SASV_flg_ovrdflg
      link override Signal_Override/_ovrdval: Value=KOUTP_SASV_flg_ovrdval
  VAPM_SNSRLayout_enum_Inproc : FVT_lib/outp/OverrideAndLimit  SystemSampleTime=-1  VariantActivationTime=update diagram  Latency=0  AutoFrameSizeCalculation=off
      link override Signal_Limit/_maxval: Value=KOUTP_SNSRLayout_enum_maxval
      link override Signal_Limit/_minval: Value=KOUTP_SNSRLayout_enum_minval
      link override Signal_Override/_ovrdflg: Value=KOUTP_SNSRLayout_enum_ovrdflg
      link override Signal_Override/_ovrdval: Value=KOUTP_SNSRLayout_enum_ovrdval
  VAPM_ShifterHandleCmdTimeOut_flg_Inproc : FVT_lib/outp/OverrideAndLimit  SystemSampleTime=-1  VariantActivationTime=update diagram  Latency=0  AutoFrameSizeCalculation=off
      link override Signal_Limit/_maxval: Value=KOUTP_ShifterHandleCmdTimeOut_flg_maxval
      link override Signal_Limit/_minval: Value=KOUTP_ShifterHandleCmdTimeOut_flg_minval
      link override Signal_Override/_ovrdflg: Value=KOUTP_ShifterHandleCmdTimeOut_flg_ovrdflg
      link override Signal_Override/_ovrdval: Value=KOUTP_ShifterHandleCmdTimeOut_flg_ovrdval
  VAPM_ShifterHandleCmd_enum_Inproc : FVT_lib/outp/OverrideAndLimit  SystemSampleTime=-1  VariantActivationTime=update diagram  Latency=0  AutoFrameSizeCalculation=off
      link override Signal_Limit/_maxval: Value=KOUTP_ShifterHandleCmd_enum_maxval
      link override Signal_Limit/_minval: Value=KOUTP_ShifterHandleCmd_enum_minval
      link override Signal_Override/_ovrdflg: Value=KOUTP_ShifterHandleCmd_enum_ovrdflg
      link override Signal_Override/_ovrdval: Value=KOUTP_ShifterHandleCmd_enum_ovrdval
  VAPM_StaFSya_flg_Inproc : FVT_lib/outp/OverrideAndLimit  SystemSampleTime=-1  VariantActivationTime=update diagram  Latency=0  AutoFrameSizeCalculation=off
      link override Signal_Limit/_maxval: Value=KOUTP_StaFSya_flg_maxval
      link override Signal_Limit/_minval: Value=KOUTP_StaFSya_flg_minval
      link override Signal_Override/_ovrdflg: Value=KOUTP_StaFSya_flg_ovrdflg
      link override Signal_Override/_ovrdval: Value=KOUTP_StaFSya_flg_ovrdval
  VAPM_TCSActiveTimeOut_flg_Inproc : FVT_lib/outp/OverrideAndLimit  SystemSampleTime=-1  VariantActivationTime=update diagram  Latency=0  AutoFrameSizeCalculation=off
      link override Signal_Limit/_maxval: Value=KOUTP_TCSActiveTimeOut_flg_maxval
      link override Signal_Limit/_minval: Value=KOUTP_TCSActiveTimeOut_flg_minval
      link override Signal_Override/_ovrdflg: Value=KOUTP_TCSActiveTimeOut_flg_ovrdflg
      link override Signal_Override/_ovrdval: Value=KOUTP_TCSActiveTimeOut_flg_ovrdval
  VAPM_TCSActive_flg_Inproc : FVT_lib/outp/OverrideAndLimit  SystemSampleTime=-1  VariantActivationTime=update diagram  Latency=0  AutoFrameSizeCalculation=off
      link override Signal_Limit/_maxval: Value=KOUTP_TCSActive_flg_maxval
      link override Signal_Limit/_minval: Value=KOUTP_TCSActive_flg_minval
      link override Signal_Override/_ovrdflg: Value=KOUTP_TCSActive_flg_ovrdflg
      link override Signal_Override/_ovrdval: Value=KOUTP_TCSActive_flg_ovrdval
  VAPM_USSStaFCL_flg_Inproc : FVT_lib/outp/OverrideAndLimit  SystemSampleTime=-1  VariantActivationTime=update diagram  Latency=0  AutoFrameSizeCalculation=off
      link override Signal_Limit/_maxval: Value=KOUTP_USSStaFCL_flg_maxval
      link override Signal_Limit/_minval: Value=KOUTP_USSStaFCL_flg_minval
      link override Signal_Override/_ovrdflg: Value=KOUTP_USSStaFCL_flg_ovrdflg
      link override Signal_Override/_ovrdval: Value=KOUTP_USSStaFCL_flg_ovrdval
  VAPM_USSStaFCR_flg_Inproc : FVT_lib/outp/OverrideAndLimit  SystemSampleTime=-1  VariantActivationTime=update diagram  Latency=0  AutoFrameSizeCalculation=off
      link override Signal_Limit/_maxval: Value=KOUTP_USSStaFCR_flg_maxval
      link override Signal_Limit/_minval: Value=KOUTP_USSStaFCR_flg_minval
      link override Signal_Override/_ovrdflg: Value=KOUTP_USSStaFCR_flg_ovrdflg
      link override Signal_Override/_ovrdval: Value=KOUTP_USSStaFCR_flg_ovrdval
  VAPM_USSStaFLL_flg_Inproc : FVT_lib/outp/OverrideAndLimit  SystemSampleTime=-1  VariantActivationTime=update diagram  Latency=0  AutoFrameSizeCalculation=off
      link override Signal_Limit/_maxval: Value=KOUTP_USSStaFLL_flg_maxval
      link override Signal_Limit/_minval: Value=KOUTP_USSStaFLL_flg_minval
      link override Signal_Override/_ovrdflg: Value=KOUTP_USSStaFLL_flg_ovrdflg
      link override Signal_Override/_ovrdval: Value=KOUTP_USSStaFLL_flg_ovrdval
  VAPM_USSStaFLR_flg_Inproc : FVT_lib/outp/OverrideAndLimit  SystemSampleTime=-1  VariantActivationTime=update diagram  Latency=0  AutoFrameSizeCalculation=off
      link override Signal_Limit/_maxval: Value=KOUTP_USSStaFLR_flg_maxval
      link override Signal_Limit/_minval: Value=KOUTP_USSStaFLR_flg_minval
      link override Signal_Override/_ovrdflg: Value=KOUTP_USSStaFLR_flg_ovrdflg
      link override Signal_Override/_ovrdval: Value=KOUTP_USSStaFLR_flg_ovrdval
  VAPM_USSStaFML_flg_Inproc : FVT_lib/outp/OverrideAndLimit  SystemSampleTime=-1  VariantActivationTime=update diagram  Latency=0  AutoFrameSizeCalculation=off
      link override Signal_Limit/_maxval: Value=KOUTP_USSStaFML_flg_maxval
      link override Signal_Limit/_minval: Value=KOUTP_USSStaFML_flg_minval
      link override Signal_Override/_ovrdflg: Value=KOUTP_USSStaFML_flg_ovrdflg
      link override Signal_Override/_ovrdval: Value=KOUTP_USSStaFML_flg_ovrdval
  VAPM_USSStaFMR_flg_Inproc : FVT_lib/outp/OverrideAndLimit  SystemSampleTime=-1  VariantActivationTime=update diagram  Latency=0  AutoFrameSizeCalculation=off
      link override Signal_Limit/_maxval: Value=KOUTP_USSStaFMR_flg_maxval
      link override Signal_Limit/_minval: Value=KOUTP_USSStaFMR_flg_minval
      link override Signal_Override/_ovrdflg: Value=KOUTP_USSStaFMR_flg_ovrdflg
      link override Signal_Override/_ovrdval: Value=KOUTP_USSStaFMR_flg_ovrdval
  VAPM_USSStaRCL_flg_Inproc : FVT_lib/outp/OverrideAndLimit  SystemSampleTime=-1  VariantActivationTime=update diagram  Latency=0  AutoFrameSizeCalculation=off
      link override Signal_Limit/_maxval: Value=KOUTP_USSStaRCL_flg_maxval
      link override Signal_Limit/_minval: Value=KOUTP_USSStaRCL_flg_minval
      link override Signal_Override/_ovrdflg: Value=KOUTP_USSStaRCL_flg_ovrdflg
      link override Signal_Override/_ovrdval: Value=KOUTP_USSStaRCL_flg_ovrdval
  VAPM_USSStaRCR_flg_Inproc : FVT_lib/outp/OverrideAndLimit  SystemSampleTime=-1  VariantActivationTime=update diagram  Latency=0  AutoFrameSizeCalculation=off
      link override Signal_Limit/_maxval: Value=KOUTP_USSStaRCR_flg_maxval
      link override Signal_Limit/_minval: Value=KOUTP_USSStaRCR_flg_minval
      link override Signal_Override/_ovrdflg: Value=KOUTP_USSStaRCR_flg_ovrdflg
      link override Signal_Override/_ovrdval: Value=KOUTP_USSStaRCR_flg_ovrdval
  VAPM_USSStaRLL_flg_Inproc : FVT_lib/outp/OverrideAndLimit  SystemSampleTime=-1  VariantActivationTime=update diagram  Latency=0  AutoFrameSizeCalculation=off
      link override Signal_Limit/_maxval: Value=KOUTP_USSStaRLL_flg_maxval
      link override Signal_Limit/_minval: Value=KOUTP_USSStaRLL_flg_minval
      link override Signal_Override/_ovrdflg: Value=KOUTP_USSStaRLL_flg_ovrdflg
      link override Signal_Override/_ovrdval: Value=KOUTP_USSStaRLL_flg_ovrdval
  VAPM_USSStaRLR_flg_Inproc : FVT_lib/outp/OverrideAndLimit  SystemSampleTime=-1  VariantActivationTime=update diagram  Latency=0  AutoFrameSizeCalculation=off
      link override Signal_Limit/_maxval: Value=KOUTP_USSStaRLR_flg_maxval
      link override Signal_Limit/_minval: Value=KOUTP_USSStaRLR_flg_minval
      link override Signal_Override/_ovrdflg: Value=KOUTP_USSStaRLR_flg_ovrdflg
      link override Signal_Override/_ovrdval: Value=KOUTP_USSStaRLR_flg_ovrdval
  VAPM_USSStaRML_flg_Inproc : FVT_lib/outp/OverrideAndLimit  SystemSampleTime=-1  VariantActivationTime=update diagram  Latency=0  AutoFrameSizeCalculation=off
      link override Signal_Limit/_maxval: Value=KOUTP_USSStaRML_flg_maxval
      link override Signal_Limit/_minval: Value=KOUTP_USSStaRML_flg_minval
      link override Signal_Override/_ovrdflg: Value=KOUTP_USSStaRML_flg_ovrdflg
      link override Signal_Override/_ovrdval: Value=KOUTP_USSStaRML_flg_ovrdval
  VAPM_USSStaRMR_flg_Inproc : FVT_lib/outp/OverrideAndLimit  SystemSampleTime=-1  VariantActivationTime=update diagram  Latency=0  AutoFrameSizeCalculation=off
      link override Signal_Limit/_maxval: Value=KOUTP_USSStaRMR_flg_maxval
      link override Signal_Limit/_minval: Value=KOUTP_USSStaRMR_flg_minval
      link override Signal_Override/_ovrdflg: Value=KOUTP_USSStaRMR_flg_ovrdflg
      link override Signal_Override/_ovrdval: Value=KOUTP_USSStaRMR_flg_ovrdval
  VAPM_VehSpeedTimeOut_flg_Inproc : FVT_lib/outp/OverrideAndLimit  SystemSampleTime=-1  VariantActivationTime=update diagram  Latency=0  AutoFrameSizeCalculation=off
      link override Signal_Limit/_maxval: Value=KOUTP_VehSpeedTimeOut_flg_maxval
      link override Signal_Limit/_minval: Value=KOUTP_VehSpeedTimeOut_flg_minval
      link override Signal_Override/_ovrdflg: Value=KOUTP_VehSpeedTimeOut_flg_ovrdflg
      link override Signal_Override/_ovrdval: Value=KOUTP_VehSpeedTimeOut_flg_ovrdval
  VAPM_VehSpeed_kph_Inproc : FVT_lib/outp/OverrideAndLimit  SystemSampleTime=-1  VariantActivationTime=update diagram  Latency=0  AutoFrameSizeCalculation=off
      link override Signal_Limit/_maxval: Value=KOUTP_VehSpeed_kph_maxval
      link override Signal_Limit/_minval: Value=KOUTP_VehSpeed_kph_minval
      link override Signal_Override/_ovrdflg: Value=KOUTP_VehSpeed_kph_ovrdflg
      link override Signal_Override/_ovrdval: Value=KOUTP_VehSpeed_kph_ovrdval
  VAPM_YawRateTimeOut_flg_Inproc : FVT_lib/outp/OverrideAndLimit  SystemSampleTime=-1  VariantActivationTime=update diagram  Latency=0  AutoFrameSizeCalculation=off
      link override Signal_Limit/_maxval: Value=KOUTP_YawRateTimeOut_flg_maxval
      link override Signal_Limit/_minval: Value=KOUTP_YawRateTimeOut_flg_minval
      link override Signal_Override/_ovrdflg: Value=KOUTP_YawRateTimeOut_flg_ovrdflg
      link override Signal_Override/_ovrdval: Value=KOUTP_YawRateTimeOut_flg_ovrdval
  VAPM_YawRateVTimeOut_flg_Inproc : FVT_lib/outp/OverrideAndLimit  SystemSampleTime=-1  VariantActivationTime=update diagram  Latency=0  AutoFrameSizeCalculation=off
      link override Signal_Limit/_maxval: Value=KOUTP_YawRateVTimeOut_flg_maxval
      link override Signal_Limit/_minval: Value=KOUTP_YawRateVTimeOut_flg_minval
      link override Signal_Override/_ovrdflg: Value=KOUTP_YawRateVTimeOut_flg_ovrdflg
      link override Signal_Override/_ovrdval: Value=KOUTP_YawRateVTimeOut_flg_ovrdval
  VAPM_YawRateV_flg_Inproc : FVT_lib/outp/OverrideAndLimit  SystemSampleTime=-1  VariantActivationTime=update diagram  Latency=0  AutoFrameSizeCalculation=off
      link override Signal_Limit/_maxval: Value=KOUTP_YawRateV_flg_maxval
      link override Signal_Limit/_minval: Value=KOUTP_YawRateV_flg_minval
      link override Signal_Override/_ovrdflg: Value=KOUTP_YawRateV_flg_ovrdflg
      link override Signal_Override/_ovrdval: Value=KOUTP_YawRateV_flg_ovrdval
  VAPM_YawRate_degps_Inproc : FVT_lib/outp/OverrideAndLimit  SystemSampleTime=-1  VariantActivationTime=update diagram  Latency=0  AutoFrameSizeCalculation=off
      link override Signal_Limit/_maxval: Value=KOUTP_YawRate_degps_maxval
      link override Signal_Limit/_minval: Value=KOUTP_YawRate_degps_minval
      link override Signal_Override/_ovrdflg: Value=KOUTP_YawRate_degps_ovrdflg
      link override Signal_Override/_ovrdval: Value=KOUTP_YawRate_degps_ovrdval
  VBCM_FDCBCMBSDBuzzerCmd_flg_Inproc : FVT_lib/outp/OverrideAndLimit  SystemSampleTime=-1  VariantActivationTime=update diagram  Latency=0  AutoFrameSizeCalculation=off
      link override Signal_Limit/_maxval: Value=KOUTP_FDCBCMBSDBuzzerCmd_flg_maxval
      link override Signal_Limit/_minval: Value=KOUTP_FDCBCMBSDBuzzerCmd_flg_minval
      link override Signal_Override/_ovrdflg: Value=KOUTP_FDCBCMBSDBuzzerCmd_flg_ovrdflg
      link override Signal_Override/_ovrdval: Value=KOUTP_FDCBCMBSDBuzzerCmd_flg_ovrdval
  VBCM_FDCBCMBrakeCmd_flg_Inproc : FVT_lib/outp/OverrideAndLimit  SystemSampleTime=-1  VariantActivationTime=update diagram  Latency=0  AutoFrameSizeCalculation=off
      link override Signal_Limit/_maxval: Value=KOUTP_FDCBCMBrakeCmd_flg_maxval
      link override Signal_Limit/_minval: Value=KOUTP_FDCBCMBrakeCmd_flg_minval
      link override Signal_Override/_ovrdflg: Value=KOUTP_FDCBCMBrakeCmd_flg_ovrdflg
      link override Signal_Override/_ovrdval: Value=KOUTP_FDCBCMBrakeCmd_flg_ovrdval
  VBCM_FDCBCMCallBellCmd_flg_Inproc : FVT_lib/outp/OverrideAndLimit  SystemSampleTime=-1  VariantActivationTime=update diagram  Latency=0  AutoFrameSizeCalculation=off
      link override Signal_Limit/_maxval: Value=KOUTP_FDCBCMCallBellCmd_flg_maxval
      link override Signal_Limit/_minval: Value=KOUTP_FDCBCMCallBellCmd_flg_minval
      link override Signal_Override/_ovrdflg: Value=KOUTP_FDCBCMCallBellCmd_flg_ovrdflg
      link override Signal_Override/_ovrdval: Value=KOUTP_FDCBCMCallBellCmd_flg_ovrdval
  VBCM_FDCBCMDVRSignalLCmd_flg_Inproc : FVT_lib/outp/OverrideAndLimit  SystemSampleTime=-1  VariantActivationTime=update diagram  Latency=0  AutoFrameSizeCalculation=off
      link override Signal_Limit/_maxval: Value=KOUTP_FDCBCMDVRSignalLCmd_flg_maxval
      link override Signal_Limit/_minval: Value=KOUTP_FDCBCMDVRSignalLCmd_flg_minval
      link override Signal_Override/_ovrdflg: Value=KOUTP_FDCBCMDVRSignalLCmd_flg_ovrdflg
      link override Signal_Override/_ovrdval: Value=KOUTP_FDCBCMDVRSignalLCmd_flg_ovrdval
  VBCM_FDCBCMDVRSignalRCmd_flg_Inproc : FVT_lib/outp/OverrideAndLimit  SystemSampleTime=-1  VariantActivationTime=update diagram  Latency=0  AutoFrameSizeCalculation=off
      link override Signal_Limit/_maxval: Value=KOUTP_FDCBCMDVRSignalRCmd_flg_maxval
      link override Signal_Limit/_minval: Value=KOUTP_FDCBCMDVRSignalRCmd_flg_minval
